simulink library "outp"  (R2021b)
settings: Solver=VariableStepAuto  StartTime=0.0  StopTime=10.0  RelTol=1e-3
undefined symbols (not defined in the file or in its folder): ENUM_PMMMODE_CHARGE, ENUM_PMMMODE_IDLE, ENUM_PMMMODE_INITIALIZE, ENUM_PMMMODE_POWERDOWN, ENUM_PMMMODE_SLEEP, Left, outp, slcm, TRUE
libraries: FVT_lib x686, hcu_lib x4, simulink x1
(part 2 of 7)

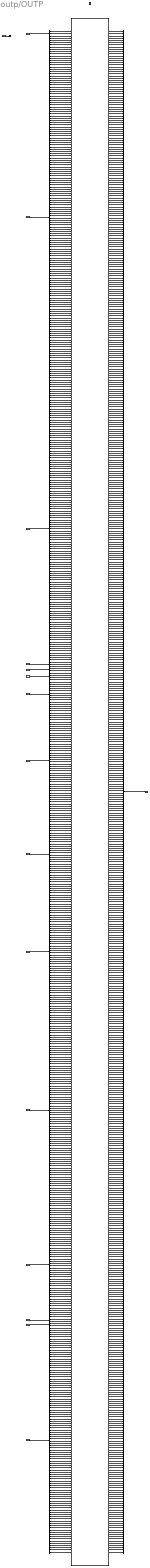
== system outp/OUTP ==
  BACC_outputs : Inport  OutDataTypeStr=Bus: BACC_outputs
  BAPM_outputs : Inport  Port=2  OutDataTypeStr=Bus: BAPM_outputs
  BBCM_outputs : Inport  Port=3  OutDataTypeStr=Bus: BBCM_outputs
  BDDM_outputs : Inport  Port=4
  BDHP_outputs : Inport  Port=5  OutDataTypeStr=Bus: BDHP_outputs
  BDKC_outputs : Inport  Port=6  OutDataTypeStr=Bus: BDKC_outputs
  BDSC_outputs : Inport  Port=7  OutDataTypeStr=Bus: BDSC_outputs
  BNMM_outputs : Inport  Port=8  OutDataTypeStr=Bus: BNMM_outputs
  BPMM_outputs : Inport  Port=9  OutDataTypeStr=Bus: BPMM_outputs
  BSYS_outputs : Inport  Port=10  OutDataTypeStr=Bus: BSYS_outputs
  BTHC_outputs : Inport  Port=11  OutDataTypeStr=Bus: BTHC_outputs
  BTPM_outputs : Inport  Port=12  OutDataTypeStr=Bus: BTPM_outputs
  BTQD_outputs : Inport  Port=13  OutDataTypeStr=Bus: BTQD_outputs
  BTQR_outputs : Inport  Port=14  OutDataTypeStr=Bus: BTQR_outputs
  BV2L_outputs : Inport  Port=15  OutDataTypeStr=Bus: BV2L_outputs
  BVMC_outputs : Inport  Port=16  OutDataTypeStr=Bus: BVMC_outputs
  trig_OUTP : TriggerPort  TriggerType=function-call  VariantControl=(inherit)
  Terminator : Terminator
  bus_creator : BusCreator  Inputs=686
  bus_selector1 : BusSelector  OutputSignals=VACC_HVTHCMSysAvail_enum,VACC_LVBattVoltSta_enum,VACC_VehHVPwrAvail4THCM_W
  bus_selector10 : BusSelector  OutputSignals=VTHC_FDCompCmd_rpm,VTHC_FDSOV1Cmd_flg,VTHC_FDSOV2Cmd_flg,VTHC_FDSOV3Cmd_flg,VTHC_FDEXV1Cmd_step,VTHC_FDEXV2Cmd_step,VTHC_FDSOTXVCmd_flg,VTHC_FDFWVCmd_flg,VTHC_FDTWVCmd_pct,VTHC_FDFrWPTCHeatPwrCmd_W,VTHC_CoolgFanActDuty_pct,VTHC_FDAGSCmd_enum,VTHC_FDEWP1Cmd_enum,VTHC_FDEWP2Cmd_enum,VTHC_FDEWP3Cmd_enum,VTHC_FDFrLeAPTCHeatPwrCmd_W,VTHC_FDFrRiAPTCHeatPwrCmd_W,VTHC_FDRrAPTCHeatPwrCmd_W,VTHC_FDBlowerCmd_pct,VTHC_BatteryMode_enum,VTHC_EDriveMode_enum,VTHC_CabinMode_enum,VTHC_CCUACLampSts_flg,VTHC_CCUAutoLampSts_flg,VTHC_CCUACMaxLampSts_flg,VTHC_CCUSyncLampSts_flg,VTHC_sigAirIntenZon1St_enum,VTHC_sigWindDirZon1St_enum,VTHC_sigRecircSt_flg,VTHC_sigSetTempZon1St_C,VTHC_sigSetTempZon2St_C,VTHC_sigClntTHvBattOut_C,VTHC_sigCbnSolarLeft_W,VTHC_sigClntTHvBattIn_C,VTHC_sigCbnSolarRight_W,VTHC_sigAmbAirT_C,VTHC_sigCbnAirT_C,VTHC_ACSubMode_enum,VTHC_FDRecyAutoCmd_enum,VTHC_ACModeMem_enum,VTHC_Face_flg,VTHC_Foot_flg,VTHC_Frost_flg,VTHC_FaceM_flg,VTHC_FootM_flg,VTHC_CCUSyncSts_flg,VTHC_ACForceOFF_flg,VTHC_RecAutoFlg_flg,VTHC_AirIntenZone1M_enum,VTHC_fdefog_flg,VTHC_sigSetTempZon2StM_C,VTHC_FDCTHCMAPTCWarningSta_flg
  bus_selector11 : BusSelector  OutputSignals=VTPM_LFBatWarn_flg,VTPM_RFBatWarn_flg,VTPM_LRBatWarn_flg,VTPM_RRBatWarn_flg,VTPM_LFWheelPress_raw8,VTPM_RFWheelPress_raw8,VTPM_LRWheelPress_raw8,VTPM_RRWheelPress_raw8,VTPM_LFWheelTemp_C,VTPM_RFWheelTemp_C,VTPM_LRWheelTemp_C,VTPM_RRWheelTemp_C,VTPM_LFSensorFail_flg,VTPM_RFSensorFail_flg,VTPM_LRSensorFail_flg,VTPM_RRSensorFail_flg,VTPM_LFWheelDebug_flg,VTPM_LRWheelDebug_flg,VTPM_RFWheelDebug_flg,VTPM_RRWheelDebug_flg,VTPM_TPMSResButtAllow_flg,VTPM_TPMSCaliButtAllow_flg,VTPM_LFPressIndi_enum,VTPM_RFPressIndi_enum,VTPM_LRPressIndi_enum,VTPM_RRPressIndi_enum,VTPM_TPMSWarnIndi_enum,VTPM_LFWheelTmpIndi_flg,VTPM_RFWheelTmpIndi_flg,VTPM_LRWheelTmpIndi_flg,VTPM_RRWheelTmpIndi_flg,VTPM_LFWheelPSW_raw8,VTPM_LRWheelPSW_raw8,VTPM_RFWheelPSW_raw8,VTPM_RRWheelPSW_raw8,VTPM_CWheelTips_enum,VTPM_AutoLTips_enum,VTPM_LFSensorMode_flg,VTPM_RFSensorMode_flg,VTPM_LRSensorMode_flg,VTPM_RRSensorMode_flg,VTPM_S1ID_raw32,VTPM_S2ID_raw32,VTPM_S3ID_raw32,VTPM_S4ID_raw32,VTPM_S1L_enum,VTPM_S2L_enum,VTPM_S3L_enum,VTPM_S4L_enum,VTPM_ALFin_flg,VTPM_LFP20_raw8,VTPM_RFP20_raw8,VTPM_LRP20_raw8,VTPM_RRP20_raw8,VTPM_FAT_flg,VTPM_IDin_raw32,VTPM_S1WheelDebugALTU_pct,VTPM_S2WheelDebugALTU_pct,VTPM_S3WheelDebugALTU_pct,VTPM_S4WheelDebugALTU_pct,VTPM_ID1messageALTU_raw8,VTPM_ID2messageALTU_raw8,VTPM_ID3messageALTU_raw8,VTPM_ID4messageALTU_raw8,VTPM_Chkfin_flg,VTPM_SetIDLoc_flg,VTPM_TPMSStorge_flg,VTPM_ChkStorge_flg,VTPM_TPMSResButt_flg,VTPM_LFPindi_enum,VTPM_RFPind_enum,VTPM_LRPindi_enum,VTPM_RRPindi_enum,VTPM_WriteChkLFID_raw,VTPM_WriteChkRFID_raw,VTPM_WriteChkLRID_raw,VTPM_WriteChkRRID_raw,VTPM_WriteChkfinLFID_raw,VTPM_WriteChkfinRFID_raw,VTPM_WriteChkfinLRID_raw,VTPM_WriteChkfinRRID_raw,VTPM_Flashchkdatavalid_enum,VTPM_Flashdatavalid_enum,VTPM_unlearnSfali_flg,VTPM_unlearnSfailvalid_enum,VTPM_Prepresstempvalid_enum,VTPM_FlashS1ID_raw,VTPM_FlashS2ID_raw,VTPM_FlashS3ID_raw,VTPM_FlashS4ID_raw,VTPM_FlashIDvalid_enum
  bus_selector12 : BusSelector  OutputSignals=VTQD_ParkRequest_flg,VTQD_TqSourceFr_enum,VTQD_TqSourceRr_enum,VTQD_FrEDUAvailBrkRgnTq_Nm,VTQD_RrEDUAvailBrkRgnTq_Nm,VTQD_EVDriveMode_enum,VTQD_ShiftGearPosn_enum,VTQD_PButtonSta_enum,VTQD_FrActvDmpDisabReq_flg,VTQD_RrActvDmpDisabReq_flg,VTQD_FrRgnDecrSta_flg,VTQD_RrRgnDecrSta_flg,VTQD_DriverWhlTqDemFr_Nm,VTQD_DriverWhlTqDemRr_Nm,VTQD_FrEDUActTq_Nm,VTQD_RrEDUActTq_Nm,VTQD_FrEDURolRgnTq_Nm,VTQD_RrEDURolRgnTq_Nm,VTQD_FrEDUSpd_rpm,VTQD_RrEDUSpd_rpm,VTQD_FrEDUSpdValid_flg,VTQD_FrEDUAvailBrkRgnTqV_flg,VTQD_RrEDUSpdValid_flg,VTQD_RrEDUAvailBrkRgnTqV_flg,VTQD_RgnAbnorSta_flg,VTQD_PTCSPermSta_flg,VTQD_FrRgnPermSta_flg,VTQD_RrRgnPermSta_flg,VTQD_FrIdcMin_A,VTQD_FrIdcMax_A,VTQD_FrUdcMin_V,VTQD_FrUdcMax_V,VTQD_RrIdcMin_A,VTQD_RrIdcMax_A,VTQD_RrUdcMin_V,VTQD_RrUdcMax_V,VTQD_ReBrakeLPReq_flg,VTQD_CreepON_flg,VTQD_EquivAccPedalSWSta_flg,VTQD_DriveProtEn_flg,VTQD_ActParkRequest_flg,VTQD_IVIPwrLockSta_enum,VTQD_OPDHoldLamp_flg,VTQD_SaveRegenMode_enum,VTQD_FDCVCURegenMode_enum,VTQD_SpdCtrlMode_enum,VTQD_SpdCtrlSta_flg,VTQD_SetSpd_kph
  bus_selector13 : BusSelector  OutputSignals=VTQR_FrTMTqReq_Nm,VTQR_RrTMTqReq_Nm
  bus_selector14 : BusSelector  OutputSignals=VV2L_ReqOBCV2LEna_enum,VV2L_ReqV2LIVIPopup_enum
  bus_selector15 : BusSelector  OutputSignals=VVMC_FeatSetSpdFinal_raw32,VVMC_VehicleSpeed_mph,VVMC_VehicleSpeed_kph,VVMC_MeterIndSpeed_raw32,VVMC_VMCAEBCtrlAvail_flg,VVMC_VMCACCCtrlAvail_flg,VVMC_VMCCCCtrlAvail_flg,VVMC_VMCMSACtrlAvail_flg,VVMC_FeatArbitrSta_enum,VVMC_FeatReqSpd_kph,VVMC_JerkPCT_pct,VVMC_LimitPCT_pct,VVMC_FrontRearSlipRatioCtrl_flg,VVMC_RearWhlSlipRatioCtrl_flg,VVMC_SingleWhlSlipRatioCtrl_flg,VVMC_LatAccCtrl_flg,VVMC_SafetyCtrl_flg,VVMC_SPD2ACCAct_flg,VVMC_AccCalcuPID_mps2,VVMC_ISOAccLimit_mps2,VVMC_ISODecLimit_mps2,VVMC_ISOJerkLimit_mps3,VVMC_ACCRequiredAccel_mps2,VVMC_DISCReqAcc_mps2,VVMC_FeatArbitrFinal_enum,VVMC_LateralCtrl_flg,VVMC_ADASLKASta_enum,VVMC_LKAStrToqReq_Nm,VVMC_LKATOIFault_flg,VVMC_LKATOIAct_enum,VVMC_ADASAEBReq_enum,VVMC_ADASFaultSta_flg,VVMC_AEBVehHoldReq_flg,VVMC_ACCVehHoldReq_flg,VVMC_ADASDBSReq_enum,VVMC_ADASACCSta_enum,VVMC_ACCObjDist_m,VVMC_ACCObjRelSpd_mps,VVMC_TimeGapLevel_enum,VVMC_ACCJerkUpperLimit_mps3,VVMC_ACCComfortBandUpper_mps2,VVMC_ACCJerkLowerLimit_mps3,VVMC_ACCComfortBandLower_mps2,VVMC_ADASVehSpdLim_raw32,VVMC_ADASShftPosnReqA_flg,VVMC_ADASShftPosnReq_enum,VVMC_ADASForceIdle_flg,VVMC_HazardWarningReq_flg,VVMC_RightTurnLightReq_flg,VVMC_LeftTurnLightReq_flg,VVMC_ADASFCWSta_enum,VVMC_ADASLDWSta_enum,VVMC_ADASFltWrnReq_flg,VVMC_ACCObjDstLvl_enum,VVMC_ForceLowBeam_enum,VVMC_ACCTakeoverReq_flg,VVMC_ADASWarningMsg_enum,VVMC_ADASCAMSpdLim_enum,VVMC_TargetType_enum,VVMC_ADASSLIFSpdLim_enum,VVMC_LKAHODDisplayWarning_flg,VVMC_LKAHODSoundWarning_flg,VVMC_ADASLFCSta_enum,VVMC_ADASLaneModeL_enum,VVMC_ADASLaneModeR_enum,VVMC_ADASSLIFSta_enum,VVMC_ADASISASta_enum,VVMC_ADASLDWMute_flg,VVMC_ADASFCWMute_flg,VVMC_ADASLFCHandsOffWarning_enum,VVMC_LVDADisabled_flg,VVMC_LVDAMuteSta_enum,VVMC_LVDAFailinfo_flg,VVMC_LVDAWarning_flg,VVMC_LVDAACCStatusInformation_flg,VVMC_ADASLFCWarnSound_enum,VVMC_FCMACCmode_enum,VVMC_ADASLanetypeR_enum,VVMC_ADASLanetypeL_enum,VVMC_ADASLanecurveL_raw32,VVMC_ADASLanecurveR_raw32,VVMC_ADASAEBSta_enum,VVMC_FCMLDWRequest_enum,VVMC_FCMLDWFault_flg,VVMC_ACCCtrlAvail_flg,VVMC_ACCPedalOvrd_flg,VVMC_TimeGapCalcu_s,VVMC_CCCtrlSta_enum,VVMC_MSACtrlSta_enum,VVMC_APSCtrlAvail_flg,VVMC_APSStaSys_enum,VVMC_APSDecReqA_flg,VVMC_APSDecReq_mps2,VVMC_APSReq_enum,VVMC_CCMSASpdWar_flg,VVMC_IMUEnaCmd_flg,VVMC_CAASCtrlAvail_flg,VVMC_CAASActive_flg,VVMC_VMCRWSActvSta_enum,VVMC_VMCRWSDfctvSta_enum,VVMC_VMCRWSPositionReq_mm,VVMC_VMCSteerFaultRequest_enum
  bus_selector2 : BusSelector  OutputSignals=VAPM_VehSpeed_kph,VAPM_VehSpeedTimeOut_flg,VAPM_FSOffSw_enum,VAPM_FSOffSwTimeOut_flg,VAPM_ChrgPlugSta_enum,VAPM_PASDRMR_cm,VAPM_PASDRML_cm,VAPM_PASDRCR_cm,VAPM_PASDRCL_cm,VAPM_PASDFMR_cm,VAPM_PASDFML_cm,VAPM_PASDFCR_cm,VAPM_PASDFCL_cm,VAPM_APSDRLR_cm,VAPM_APSDRLL_cm,VAPM_APSDFLR_cm,VAPM_APSDFLL_cm,VAPM_PASAFCL_enum,VAPM_PASARMR_enum,VAPM_PASARML_enum,VAPM_PASARCR_enum,VAPM_PASARCL_enum,VAPM_PASAFMR_enum,VAPM_PASAFML_enum,VAPM_PASAFCR_enum,VAPM_USSStaRMR_flg,VAPM_USSStaRML_flg,VAPM_USSStaRLR_flg,VAPM_USSStaRLL_flg,VAPM_USSStaRCR_flg,VAPM_USSStaRCL_flg,VAPM_USSStaFMR_flg,VAPM_USSStaFML_flg,VAPM_USSStaFLR_flg,VAPM_USSStaFLL_flg,VAPM_USSStaFCR_flg,VAPM_USSStaFCL_flg,VAPM_Chime_enum,VAPM_SNSRLayout_enum,VAPM_StaFSya_flg,VAPM_ModOperation_enum,VAPM_BrkPedalPos_pct,VAPM_BrkPedalPosTimeOut_flg,VAPM_LFRawWhlSpeed_kph,VAPM_LFRawWhlSpeedTimeOut_flg,VAPM_RFRawWhlSpeed_kph,VAPM_RFRawWhlSpeedTimeOut_flg,VAPM_LRRawWhlSpeed_kph,VAPM_LRRawWhlSpeedTimeOut_flg,VAPM_RRRawWhlSpeed_kph,VAPM_RRRawWhlSpeedTimeOut_flg,VAPM_LFRawWhlSpeedV_flg,VAPM_LFRawWhlSpeedVTimeOut_flg,VAPM_RFRawWhlSpeedV_flg,VAPM_RFRawWhlSpeedVTimeOut_flg,VAPM_LRRawWhlSpeedV_flg,VAPM_LRRawWhlSpeedVTimeOut_flg,VAPM_RRRawWhlSpeedV_flg,VAPM_RRRawWhlSpeedVTimeOut_flg,VAPM_LFWhlRotDir_enum,VAPM_LFWhlRotDirTimeOut_flg,VAPM_RFWhlRotDir_enum,VAPM_RFWhlRotDirTimeOut_flg,VAPM_LRWhlRotDir_enum,VAPM_LRWhlRotDirTimeOut_flg,VAPM_RRWhlRotDir_enum,VAPM_RRWhlRotDirTimeOut_flg,VAPM_LFPulseCountV_flg,VAPM_LFPulseCountVTimeOut_flg,VAPM_RFPulseCountV_flg,VAPM_RFPulseCountVTimeOut_flg,VAPM_LRPulseCountV_flg,VAPM_LRPulseCountVTimeOut_flg,VAPM_RRPulseCountV_flg,VAPM_RRPulseCountVTimeOut_flg,VAPM_LFPulseCount_enum,VAPM_LFPulseCountTimeOut_flg,VAPM_RFPulseCount_enum,VAPM_RFPulseCountTimeOut_flg,VAPM_LRPulseCount_enum,VAPM_LRPulseCountTimeOut_flg,VAPM_RRPulseCount_enum,VAPM_RRPulseCountTimeOut_flg,VAPM_ShifterHandleCmd_enum,VAPM_ShifterHandleCmdTimeOut_flg,VAPM_DriIntend_enum,VAPM_DriIntendTimeOut_flg,VAPM_EPSAOIControl_enum,VAPM_EPSAOIControlTimeOut_flg,VAPM_SASAngle_Deg,VAPM_SASAngleTimeOut_flg,VAPM_SASSpeed_degps,VAPM_SASSpeedTimeOut_flg,VAPM_SASSpeedValid_flg,VAPM_SASSpeedValidTimeOut_flg,VAPM_SASCAL_flg,VAPM_SASCALTimeOut_flg,VAPM_SASV_flg,VAPM_SASVTimeOut_flg,VAPM_GRADE_Deg,VAPM_GRADETimeOut_flg,VAPM_YawRate_degps,VAPM_YawRateTimeOut_flg,VAPM_LatAccel_Gps,VAPM_LatAccelTimeOut_flg,VAPM_LongAccel_Gps,VAPM_LongAccelTimeOut_flg,VAPM_MCPressure_bar,VAPM_MCPressureTimeOut_flg,VAPM_YawRateV_flg,VAPM_YawRateVTimeOut_flg,VAPM_LatAccelV_flg,VAPM_LatAccelVTimeOut_flg,VAPM_LongAccelV_flg,VAPM_LongAccelVTimeOut_flg,VAPM_MCPressureV_bar,VAPM_MCPressureVTimeOut_flg,VAPM_BrkSwSta_flg,VAPM_BrkSwStaTimeOut_flg,VAPM_BrkSwV_flg,VAPM_BrkSwVTimeOut_flg,VAPM_ESCStandstill_flg,VAPM_ESCStandstillTimeOut_flg,VAPM_ESCAPSSta_enum,VAPM_ESCAPSStaTimeOut_flg,VAPM_EPBExtReleaseAvail_flg,VAPM_EPBExtReleaseAvailTimeOut_flg,VAPM_EPBExtApplyAvail_flg,VAPM_EPBExtApplyAvailTimeOut_flg,VAPM_EPBErrSta_enum,VAPM_EPBErrStaTimeOut_flg,VAPM_EPBSta_enum,VAPM_EPBStaTimeOut_flg,VAPM_AVMparkingcancel_enum,VAPM_AVMparkingcancelTimeOut_flg,VAPM_AVMparkingexcute_enum,VAPM_AVMparkingexcuteTimeOut_flg,VAPM_AVMParkingmode_enum,VAPM_AVMParkingmodeTimeOut_flg,VAPM_AVMErrSTA_flg,VAPM_AVMErrSTATimeOut_flg,VAPM_IVIStatus_flg,VAPM_IVIStatusTimeOut_flg,VAPM_CAASSw_enum,VAPM_CAASSwTimeOut_flg,VAPM_IVIScreen_enum,VAPM_IVIScreenTimeOut_flg,VAPM_ABSActive_flg,VAPM_ABSActiveTimeOut_flg,VAPM_TCSActive_flg,VAPM_TCSActiveTimeOut_flg,VAPM_DriverSeatBeltCmd_flg,VAPM_DriverSeatBeltCmdTimeOut_flg,VAPM_APSProgressPCT_pct,VAPM_APSRQDisplay_enum,VAPM_APSSWVer_enum,VAPM_APSHWVer_enum,VAPM_APSExitCondition_enum,VAPM_APSAngleTarget_Deg,VAPM_APSVRqEPASCtrl_flg,VAPM_APSRqEPASCtrl_flg,VAPM_CAASSta_enum
  bus_selector3 : BusSelector  OutputSignals=VBCM_AntitheftSta_enum,VBCM_TailgateRemote_enum,VBCM_HornCtrl_flg,VBCM_AllDoorSW_flg,VBCM_BCMDoorLockSta_flg,VBCM_AntitheftSeatFlod_flg,VBCM_HoodSW_flg,VBCM_TailgateSW_flg,VBCM_DrDoorSW_flg,VBCM_PsDoorSW_flg,VBCM_RLDoorSW_flg,VBCM_RRDoorSW_flg,VBCM_LockSetting_flg,VBCM_FrChargingDoorCtrl_enum,VBCM_RrChargingDoorCtrl_enum,VBCM_CrashDetd_flg,VBCM_CTDCtrl_enum,VBCM_DoorLockIND_flg,VBCM_CTDLockSW_flg,VBCM_Dimmer_pct,VBCM_DimmerEN_flg,VBCM_PosLamp_flg,VBCM_LBeam_flg,VBCM_HBeam_flg,VBCM_RrFogLamp_flg,VBCM_BrakeLamp_flg,VBCM_ReverseLamp_flg,VBCM_LDRL_flg,VBCM_RDRL_flg,VBCM_LBSD_flg,VBCM_RBSD_flg,VBCM_HazardSW_flg,VBCM_LTurnLP_flg,VBCM_RTurnLP_flg,VBCM_BCMBuzzerReq_flg,VBCM_MirrorCtrl_enum,VBCM_MirrorDefog_flg,VBCM_RrDefog_flg,VBCM_RoomLampH_flg,VBCM_RoomLampL_flg,VBCM_TrunkRel_flg,VBCM_TailgateHDSW_flg,VBCM_FrWiperL_flg,VBCM_FrWiperH_flg,VBCM_RrWiper_flg,VBCM_WasherCtrl_enum,VBCM_WiperFixMode_flg,VBCM_AmbLightBreath1_enum,VBCM_AmbLightBreath2_enum,VBCM_AmbLightBreath3_enum,VBCM_AmbLightBreath4_enum,VBCM_AmbLightBreath5_enum,VBCM_AmbLightBreath6_enum,VBCM_AmbLightBrightness1_enum,VBCM_AmbLightBrightness2_enum,VBCM_AmbLightBrightness3_enum,VBCM_AmbLightBrightness4_enum,VBCM_AmbLightBrightness5_enum,VBCM_AmbLightBrightness6_enum,VBCM_AmbLightColor1_enum,VBCM_AmbLightColor2_enum,VBCM_AmbLightColor3_enum,VBCM_AmbLightColor4_enum,VBCM_AmbLightColor5_enum,VBCM_AmbLightColor6_enum,VBCM_LampPwr_flg,VBCM_SPTGDet_flg,VBCM_APSOpenPTG_flg,VBCM_FollowMe_flg,VBCM_IVIRST_flg,VBCM_CountAlarm_enum,VBCM_MFSWTri_flg,VBCM_MirrorFlodPos_flg,VBCM_FuelDoorPos_flg,VBCM_MFRDNBrightReq_pct,VBCM_RoomLampMode_flg,VBCM_IVIPTGUSStaSW_flg,VBCM_PTGInnerSW2_enum,VBCM_LDrvCtrlCmd_pct,VBCM_LPasCtrlCmd_pct,VBCM_LRLDCtrlCmd_pct,VBCM_LRRDCtrlCmd_pct,VBCM_APMDoorControlSta_flg,VBCM_AmbFunEN_flg,VBCM_AmbWelEN_flg,VBCM_AmbDimEN_flg,VBCM_AmbLinkDriSta_flg,VBCM_AmbPwrWarnEN_flg,VBCM_AmbODAEN_flg,VBCM_AmbColorSta_enum,VBCM_AmbBrightSta_enum,VBCM_LockAlarm_enum,VBCM_ATCtrl_enum,VBCM_fUnlockSingle_flg,VBCM_UserNow_enum,VBCM_AmbFunENFlash_enum,VBCM_AmbWelENFlash_enum,VBCM_AmbDimENFlash_enum,VBCM_AmbLinkDriStaFlash_enum,VBCM_AmbPwrWarnENFlash_enum,VBCM_AmbODAENFlash_enum,VBCM_AmbColorSta1_enum,VBCM_AmbColorSta2_enum,VBCM_AmbColorSta3_enum,VBCM_AmbColorSta4_enum,VBCM_AmbColorSta5_enum,VBCM_AmbColorSta7_enum,VBCM_AmbBrightnessSta1_enum,VBCM_AmbBrightnessSta2_enum,VBCM_AmbBrightnessSta3_enum,VBCM_AmbBrightnessSta4_enum,VBCM_AmbBrightnessSta5_enum,VBCM_AmbBrightnessSta7_enum,VBCM_HazardIND_flg,VBCM_DimSwSta_flg,VBCM_PassSWSta_flg,VBCM_FWipSwSta_enum,VBCM_FWasSwSta_enum,VBCM_TurnSwSta_enum
  bus_selector4 : BusSelector  OutputSignals=VDHP_ActAPSPosn_pct,VDHP_EAPS1MIN_pct,VDHP_EAPS2MIN_pct
  bus_selector5 : BusSelector  OutputSignals=VDKC_DKCTimeSN_cnt,VDKC_DKCAuthSta_enum
  bus_selector6 : BusSelector  OutputSignals=VDSC_DISCTurn_flg,VDSC_DISCTargetSpd_kph,VDSC_DISCSta_enum,VDSC_DISCButtSta_flg
  bus_selector7 : BusSelector  OutputSignals=VNMM_AllCANTxReq_flg,VNMM_NMmTxReq_flg,VNMM_Awake_enum,VNMM_CSB_flg,VNMM_ErrorState_enum,VNMM_NodeID_enum,VNMM_PNI_flg,VNMM_RptMsgReq_flg,VNMM_WakeUp_enum,VNMM_ActiveWU_flg,VNMM_SysNMmSta_enum,VNMM_NetworkReq_flg
  bus_selector8 : BusSelector  OutputSignals=VPMM_PowerUpState_enum,VPMM_PowerDownState_enum,VPMM_PowerUpFault_enum,VPMM_PowerDownFault_enum,VPMM_ActiveDischargeReq_flg,VPMM_DCDCEnaReq_flg,VPMM_DCDCVoltSetpoint_V,VPMM_HVBatCnctReq_flg,VPMM_HVSysReadyToCharge_enum,VPMM_PowerSta_enum,VPMM_LVPwrSta_flg,VPMM_HVPwrSta_flg,VPMM_SysPowerMode_enum,VPMM_FrMCUEnaReq_flg,VPMM_RrMCUEnaReq_flg,VPMM_DrivetrainSelect_enum,VPMM_DrSeatSta_enum,VPMM_PwrStaSelect_enum,VPMM_PwrStaConstraint_enum,VPMM_TCountSta_enum,VPMM_PwrUpReq_enum,VPMM_PwrDownReq_enum,VPMM_LowSOCWarn_enum,VPMM_ReVehThdChkSta_enum,VPMM_LVSysErrPwrOutErr_flg,VPMM_EvccAplusPwrUpReq_flg,VPMM_PwrStaONTOPopReq_flg,VPMM_IVIPwrStaONTOPopT_s,VPMM_LVChrgHoldTtimer_s,VPMM_LVBattChrgTimeCnt_s,VPMM_SilentChkAllowSleep_flg,VPMM_TimerAllowSleep_flg,VPMM_FDADC12VDetAvg_mV,VPMM_PMMAllowECUSleep_flg,VPMM_LVSilentChrgSta_enum,VPMM_LVSilentChrgReq_flg,VPMM_LVSilentChrgLv_enum,VPMM_CtrlFrPwrStbA1P_flg,VPMM_CtrlFrRC1_flg,VPMM_CtrlFrBMSCCUCIR_flg,VPMM_CtrlFrEDUINVERTER_flg,VPMM_HWResetSta_enum,VPMM_CtrlDrPwrStbA2_flg,VPMM_PwrStaTOSta_enum,VPMM_Sched_ChgTOSta_enum,VPMM_PwrReq_OTA_enum,VPMM_OTAPwrReqOFFChkSta_enum,VPMM_OTAPwrReqStdChkSta_enum
  bus_selector9 : BusSelector  OutputSignals=VSYS_HWVer1_cnt,VSYS_HWVer2_cnt,VSYS_HWVer3_cnt,VSYS_CarModel1_cnt,VSYS_CarModel2_cnt,VSYS_CarModel3_cnt,VSYS_ECU1_cnt,VSYS_ECU2_cnt,VSYS_Major1_cnt,VSYS_Major2_cnt,VSYS_Minor1_cnt,VSYS_Minor2_cnt,VSYS_Patch1_cnt,VSYS_Patch2_cnt,VSYS_Country1_cnt,VSYS_Country2_cnt,VSYS_Variation_cnt,VSYS_Dash1_cnt,VSYS_Change1_cnt,VSYS_Change2_cnt,VSYS_Dash2_cnt,VSYS_SHA1_cnt,VSYS_SHA2_cnt,VSYS_SHA3_cnt,VSYS_SHA4_cnt,VSYS_SHA5_cnt,VSYS_SHA6_cnt,VSYS_SHA7_cnt,VSYS_SHA8_cnt,VSYS_NvWriteReqRisingEdge_flg,VSYS_FdcSlpReqRisingEdge_flg,VSYS_FdcSlpTime_sec,VSYS_PmicBootReason_enum,VSYS_WisrBootReason_raw32,VSYS_AcoreRebootCmdACK_flg,VSYS_CurrentNmState_enum
  outpmodule : Subsystem
  BOUTP_outputs : Outport  OutDataTypeStr=Bus: BOUTP_outputs
  wires:
  BDDM_outputs/1 -> Terminator/1
  outpmodule/92(VOUTP_EPSAOIControlTimeOut_flg) -> bus_creator/92
  outpmodule/91(VOUTP_EPSAOIControl_enum) -> bus_creator/91
  outpmodule/90(VOUTP_DriIntendTimeOut_flg) -> bus_creator/90
  outpmodule/117(VOUTP_LongAccelV_flg) -> bus_creator/117
  outpmodule/87(VOUTP_ShifterHandleCmd_enum) -> bus_creator/87
  bus_selector15/101 -> outpmodule/685(VVMC_VMCRWSPositionReq_mm)  "<VVMC_VMCRWSPositionReq_mm>"
  bus_selector15/102 -> outpmodule/686(VVMC_VMCSteerFaultRequest_enum)  "<VVMC_VMCSteerFaultRequest_enum>"
  bus_selector15/100 -> outpmodule/684(VVMC_VMCRWSDfctvSta_enum)  "<VVMC_VMCRWSDfctvSta_enum>"
  outpmodule/97(VOUTP_SASSpeedValid_flg) -> bus_creator/97
  bus_selector15/97 -> outpmodule/681(VVMC_CAASCtrlAvail_flg)  "<VVMC_CAASCtrlAvail_flg>"
  bus_selector15/95 -> outpmodule/679(VVMC_CCMSASpdWar_flg)  "<VVMC_CCMSASpdWar_flg>"
  bus_selector15/94 -> outpmodule/678(VVMC_APSReq_enum)  "<VVMC_APSReq_enum>"
  bus_selector15/92 -> outpmodule/676(VVMC_APSDecReqA_flg)  "<VVMC_APSDecReqA_flg>"
  bus_selector15/89 -> outpmodule/673(VVMC_MSACtrlSta_enum)  "<VVMC_MSACtrlSta_enum>"
  bus_selector15/86 -> outpmodule/670(VVMC_ACCPedalOvrd_flg)  "<VVMC_ACCPedalOvrd_flg>"
  bus_selector15/85 -> outpmodule/669(VVMC_ACCCtrlAvail_flg)  "<VVMC_ACCCtrlAvail_flg>"
  bus_selector15/79 -> outpmodule/663(VVMC_ADASLanetypeL_enum)  "<VVMC_ADASLanetypeL_enum>"
  bus_selector15/80 -> outpmodule/664(VVMC_ADASLanecurveL_raw32)  "<VVMC_ADASLanecurveL_raw32>"
  bus_selector15/78 -> outpmodule/662(VVMC_ADASLanetypeR_enum)  "<VVMC_ADASLanetypeR_enum>"
  bus_selector15/77 -> outpmodule/661(VVMC_FCMACCmode_enum)  "<VVMC_FCMACCmode_enum>"
  bus_selector15/76 -> outpmodule/660(VVMC_ADASLFCWarnSound_enum)  "<VVMC_ADASLFCWarnSound_enum>"
  bus_selector15/75 -> outpmodule/659(VVMC_LVDAACCStatusInformation_flg)  "<VVMC_LVDAACCStatusInformation_flg>"
  bus_selector15/74 -> outpmodule/658(VVMC_LVDAWarning_flg)  "<VVMC_LVDAWarning_flg>"
  bus_selector15/69 -> outpmodule/653(VVMC_ADASFCWMute_flg)  "<VVMC_ADASFCWMute_flg>"
  bus_selector15/67 -> outpmodule/651(VVMC_ADASISASta_enum)  "<VVMC_ADASISASta_enum>"
  bus_selector15/66 -> outpmodule/650(VVMC_ADASSLIFSta_enum)  "<VVMC_ADASSLIFSta_enum>"
  bus_selector15/65 -> outpmodule/649(VVMC_ADASLaneModeR_enum)  "<VVMC_ADASLaneModeR_enum>"
  outpmodule/95(VOUTP_SASSpeed_degps) -> bus_creator/95
  bus_selector15/63 -> outpmodule/647(VVMC_ADASLFCSta_enum)  "<VVMC_ADASLFCSta_enum>"
  bus_selector15/60 -> outpmodule/644(VVMC_ADASSLIFSpdLim_enum)  "<VVMC_ADASSLIFSpdLim_enum>"
  bus_selector15/59 -> outpmodule/643(VVMC_TargetType_enum)  "<VVMC_TargetType_enum>"
  bus_selector15/55 -> outpmodule/639(VVMC_ForceLowBeam_enum)  "<VVMC_ForceLowBeam_enum>"
  bus_selector15/51 -> outpmodule/635(VVMC_ADASFCWSta_enum)  "<VVMC_ADASFCWSta_enum>"
  bus_selector15/53 -> outpmodule/637(VVMC_ADASFltWrnReq_flg)  "<VVMC_ADASFltWrnReq_flg>"
  bus_selector15/52 -> outpmodule/636(VVMC_ADASLDWSta_enum)  "<VVMC_ADASLDWSta_enum>"
  bus_selector15/50 -> outpmodule/634(VVMC_LeftTurnLightReq_flg)  "<VVMC_LeftTurnLightReq_flg>"
  bus_selector15/49 -> outpmodule/633(VVMC_RightTurnLightReq_flg)  "<VVMC_RightTurnLightReq_flg>"
  bus_selector15/48 -> outpmodule/632(VVMC_HazardWarningReq_flg)  "<VVMC_HazardWarningReq_flg>"
  bus_selector15/73 -> outpmodule/657(VVMC_LVDAFailinfo_flg)  "<VVMC_LVDAFailinfo_flg>"
  bus_selector15/46 -> outpmodule/630(VVMC_ADASShftPosnReq_enum)  "<VVMC_ADASShftPosnReq_enum>"
  bus_selector15/43 -> outpmodule/627(VVMC_ACCComfortBandLower_mps2)  "<VVMC_ACCComfortBandLower_mps2>"
  bus_selector15/41 -> outpmodule/625(VVMC_ACCComfortBandUpper_mps2)  "<VVMC_ACCComfortBandUpper_mps2>"
  bus_selector15/42 -> outpmodule/626(VVMC_ACCJerkLowerLimit_mps3)  "<VVMC_ACCJerkLowerLimit_mps3>"
  outpmodule/93(VOUTP_SASAngle_Deg) -> bus_creator/93
  bus_selector15/29 -> outpmodule/613(VVMC_LKATOIFault_flg)  "<VVMC_LKATOIFault_flg>"
  bus_selector15/19 -> outpmodule/603(VVMC_AccCalcuPID_mps2)  "<VVMC_AccCalcuPID_mps2>"
  bus_selector15/17 -> outpmodule/601(VVMC_SafetyCtrl_flg)  "<VVMC_SafetyCtrl_flg>"
  bus_selector15/18 -> outpmodule/602(VVMC_SPD2ACCAct_flg)  "<VVMC_SPD2ACCAct_flg>"
  bus_selector15/33 -> outpmodule/617(VVMC_AEBVehHoldReq_flg)  "<VVMC_AEBVehHoldReq_flg>"
  bus_selector15/15 -> outpmodule/599(VVMC_SingleWhlSlipRatioCtrl_flg)  "<VVMC_SingleWhlSlipRatioCtrl_flg>"
  bus_selector15/14 -> outpmodule/598(VVMC_RearWhlSlipRatioCtrl_flg)  "<VVMC_RearWhlSlipRatioCtrl_flg>"
  bus_selector15/37 -> outpmodule/621(VVMC_ACCObjDist_m)  "<VVMC_ACCObjDist_m>"
  bus_selector15/13 -> outpmodule/597(VVMC_FrontRearSlipRatioCtrl_flg)  "<VVMC_FrontRearSlipRatioCtrl_flg>"
  bus_selector15/12 -> outpmodule/596(VVMC_LimitPCT_pct)  "<VVMC_LimitPCT_pct>"
  bus_selector15/10 -> outpmodule/594(VVMC_FeatReqSpd_kph)  "<VVMC_FeatReqSpd_kph>"
  bus_selector15/8 -> outpmodule/592(VVMC_VMCMSACtrlAvail_flg)  "<VVMC_VMCMSACtrlAvail_flg>"
  bus_selector15/11 -> outpmodule/595(VVMC_JerkPCT_pct)  "<VVMC_JerkPCT_pct>"
  bus_selector15/32 -> outpmodule/616(VVMC_ADASFaultSta_flg)  "<VVMC_ADASFaultSta_flg>"
  bus_selector15/5 -> outpmodule/589(VVMC_VMCAEBCtrlAvail_flg)  "<VVMC_VMCAEBCtrlAvail_flg>"
  bus_selector15/9 -> outpmodule/593(VVMC_FeatArbitrSta_enum)  "<VVMC_FeatArbitrSta_enum>"
  bus_selector15/1 -> outpmodule/585(VVMC_FeatSetSpdFinal_raw32)  "<VVMC_FeatSetSpdFinal_raw32>"
  bus_selector14/1 -> outpmodule/583(VV2L_ReqOBCV2LEna_enum)  "<VV2L_ReqOBCV2LEna_enum>"
  BV2L_outputs/1 -> bus_selector14/1
  bus_selector13/1 -> outpmodule/581(VTQR_FrTMTqReq_Nm)  "<VTQR_FrTMTqReq_Nm>"
  BTQD_outputs/1 -> bus_selector12/1
  bus_selector13/2 -> outpmodule/582(VTQR_RrTMTqReq_Nm)  "<VTQR_RrTMTqReq_Nm>"
  bus_selector12/48 -> outpmodule/580(VTQD_SetSpd_kph)  "<VTQD_SetSpd_kph>"
  bus_selector12/47 -> outpmodule/579(VTQD_SpdCtrlSta_flg)  "<VTQD_SpdCtrlSta_flg>"
  bus_selector12/42 -> outpmodule/574(VTQD_IVIPwrLockSta_enum)  "<VTQD_IVIPwrLockSta_enum>"
  bus_selector12/43 -> outpmodule/575(VTQD_OPDHoldLamp_flg)  "<VTQD_OPDHoldLamp_flg>"
  bus_selector11/32 -> outpmodule/473(VTPM_LFWheelPSW_raw8)  "<VTPM_LFWheelPSW_raw8>"
  bus_selector11/31 -> outpmodule/472(VTPM_RRWheelTmpIndi_flg)  "<VTPM_RRWheelTmpIndi_flg>"
  bus_selector11/30 -> outpmodule/471(VTPM_LRWheelTmpIndi_flg)  "<VTPM_LRWheelTmpIndi_flg>"
  bus_selector11/46 -> outpmodule/487(VTPM_S1L_enum)  "<VTPM_S1L_enum>"
  bus_selector11/29 -> outpmodule/470(VTPM_RFWheelTmpIndi_flg)  "<VTPM_RFWheelTmpIndi_flg>"
  bus_selector11/27 -> outpmodule/468(VTPM_TPMSWarnIndi_enum)  "<VTPM_TPMSWarnIndi_enum>"
  BTHC_outputs/1 -> bus_selector10/1
  bus_selector10/51 -> outpmodule/440(VTHC_sigSetTempZon2StM_C)  "<VTHC_sigSetTempZon2StM_C>"
  bus_selector10/52 -> outpmodule/441(VTHC_FDCTHCMAPTCWarningSta_flg)  "<VTHC_FDCTHCMAPTCWarningSta_flg>"
  bus_selector10/50 -> outpmodule/439(VTHC_fdefog_flg)  "<VTHC_fdefog_flg>"
  bus_selector10/49 -> outpmodule/438(VTHC_AirIntenZone1M_enum)  "<VTHC_AirIntenZone1M_enum>"
  bus_selector10/47 -> outpmodule/436(VTHC_ACForceOFF_flg)  "<VTHC_ACForceOFF_flg>"
  bus_selector10/45 -> outpmodule/434(VTHC_FootM_flg)  "<VTHC_FootM_flg>"
  bus_selector10/46 -> outpmodule/435(VTHC_CCUSyncSts_flg)  "<VTHC_CCUSyncSts_flg>"
  bus_selector10/43 -> outpmodule/432(VTHC_Frost_flg)  "<VTHC_Frost_flg>"
  bus_selector10/40 -> outpmodule/429(VTHC_ACModeMem_enum)  "<VTHC_ACModeMem_enum>"
  bus_selector10/44 -> outpmodule/433(VTHC_FaceM_flg)  "<VTHC_FaceM_flg>"
  bus_selector10/42 -> outpmodule/431(VTHC_Foot_flg)  "<VTHC_Foot_flg>"
  bus_selector10/37 -> outpmodule/426(VTHC_sigCbnAirT_C)  "<VTHC_sigCbnAirT_C>"
  bus_selector10/35 -> outpmodule/424(VTHC_sigCbnSolarRight_W)  "<VTHC_sigCbnSolarRight_W>"
  bus_selector10/34 -> outpmodule/423(VTHC_sigClntTHvBattIn_C)  "<VTHC_sigClntTHvBattIn_C>"
  bus_selector10/32 -> outpmodule/421(VTHC_sigClntTHvBattOut_C)  "<VTHC_sigClntTHvBattOut_C>"
  bus_selector10/33 -> outpmodule/422(VTHC_sigCbnSolarLeft_W)  "<VTHC_sigCbnSolarLeft_W>"
  bus_selector10/31 -> outpmodule/420(VTHC_sigSetTempZon2St_C)  "<VTHC_sigSetTempZon2St_C>"
  bus_selector10/30 -> outpmodule/419(VTHC_sigSetTempZon1St_C)  "<VTHC_sigSetTempZon1St_C>"
  bus_selector10/28 -> outpmodule/417(VTHC_sigWindDirZon1St_enum)  "<VTHC_sigWindDirZon1St_enum>"
  bus_selector10/27 -> outpmodule/416(VTHC_sigAirIntenZon1St_enum)  "<VTHC_sigAirIntenZon1St_enum>"
  bus_selector10/24 -> outpmodule/413(VTHC_CCUAutoLampSts_flg)  "<VTHC_CCUAutoLampSts_flg>"
  bus_selector10/26 -> outpmodule/415(VTHC_CCUSyncLampSts_flg)  "<VTHC_CCUSyncLampSts_flg>"
  bus_selector10/25 -> outpmodule/414(VTHC_CCUACMaxLampSts_flg)  "<VTHC_CCUACMaxLampSts_flg>"
  bus_selector10/23 -> outpmodule/412(VTHC_CCUACLampSts_flg)  "<VTHC_CCUACLampSts_flg>"
  bus_selector10/22 -> outpmodule/411(VTHC_CabinMode_enum)  "<VTHC_CabinMode_enum>"
  bus_selector10/21 -> outpmodule/410(VTHC_EDriveMode_enum)  "<VTHC_EDriveMode_enum>"
  bus_selector10/19 -> outpmodule/408(VTHC_FDBlowerCmd_pct)  "<VTHC_FDBlowerCmd_pct>"
  bus_selector10/15 -> outpmodule/404(VTHC_FDEWP3Cmd_enum)  "<VTHC_FDEWP3Cmd_enum>"
  bus_selector10/12 -> outpmodule/401(VTHC_FDAGSCmd_enum)  "<VTHC_FDAGSCmd_enum>"
  bus_selector10/13 -> outpmodule/402(VTHC_FDEWP1Cmd_enum)  "<VTHC_FDEWP1Cmd_enum>"
  bus_selector10/10 -> outpmodule/399(VTHC_FDFrWPTCHeatPwrCmd_W)  "<VTHC_FDFrWPTCHeatPwrCmd_W>"
  bus_selector10/8 -> outpmodule/397(VTHC_FDFWVCmd_flg)  "<VTHC_FDFWVCmd_flg>"
  bus_selector10/6 -> outpmodule/395(VTHC_FDEXV2Cmd_step)  "<VTHC_FDEXV2Cmd_step>"
  bus_selector10/16 -> outpmodule/405(VTHC_FDFrLeAPTCHeatPwrCmd_W)  "<VTHC_FDFrLeAPTCHeatPwrCmd_W>"
  bus_selector11/37 -> outpmodule/478(VTPM_AutoLTips_enum)  "<VTPM_AutoLTips_enum>"
  bus_selector10/4 -> outpmodule/393(VTHC_FDSOV3Cmd_flg)  "<VTHC_FDSOV3Cmd_flg>"
  bus_selector10/3 -> outpmodule/392(VTHC_FDSOV2Cmd_flg)  "<VTHC_FDSOV2Cmd_flg>"
  bus_selector11/24 -> outpmodule/465(VTPM_RFPressIndi_enum)  "<VTPM_RFPressIndi_enum>"
  bus_selector11/22 -> outpmodule/463(VTPM_TPMSCaliButtAllow_flg)  "<VTPM_TPMSCaliButtAllow_flg>"
  bus_selector11/21 -> outpmodule/462(VTPM_TPMSResButtAllow_flg)  "<VTPM_TPMSResButtAllow_flg>"
  bus_selector11/18 -> outpmodule/459(VTPM_LRWheelDebug_flg)  "<VTPM_LRWheelDebug_flg>"
  bus_selector11/17 -> outpmodule/458(VTPM_LFWheelDebug_flg)  "<VTPM_LFWheelDebug_flg>"
  bus_selector11/16 -> outpmodule/457(VTPM_RRSensorFail_flg)  "<VTPM_RRSensorFail_flg>"
  bus_selector11/15 -> outpmodule/456(VTPM_LRSensorFail_flg)  "<VTPM_LRSensorFail_flg>"
  bus_selector11/10 -> outpmodule/451(VTPM_RFWheelTemp_C)  "<VTPM_RFWheelTemp_C>"
  bus_selector11/9 -> outpmodule/450(VTPM_LFWheelTemp_C)  "<VTPM_LFWheelTemp_C>"
  bus_selector11/7 -> outpmodule/448(VTPM_LRWheelPress_raw8)  "<VTPM_LRWheelPress_raw8>"
  bus_selector11/8 -> outpmodule/449(VTPM_RRWheelPress_raw8)  "<VTPM_RRWheelPress_raw8>"
  bus_selector11/6 -> outpmodule/447(VTPM_RFWheelPress_raw8)  "<VTPM_RFWheelPress_raw8>"
  bus_selector11/39 -> outpmodule/480(VTPM_RFSensorMode_flg)  "<VTPM_RFSensorMode_flg>"
  bus_selector11/3 -> outpmodule/444(VTPM_LRBatWarn_flg)  "<VTPM_LRBatWarn_flg>"
  bus_selector11/4 -> outpmodule/445(VTPM_RRBatWarn_flg)  "<VTPM_RRBatWarn_flg>"
  bus_selector11/1 -> outpmodule/442(VTPM_LFBatWarn_flg)  "<VTPM_LFBatWarn_flg>"
  bus_selector11/26 -> outpmodule/467(VTPM_RRPressIndi_enum)  "<VTPM_RRPressIndi_enum>"
  bus_selector2/14 -> outpmodule/17(VAPM_APSDRLR_cm)  "<VAPM_APSDRLR_cm>"
  bus_selector2/2 -> outpmodule/5(VAPM_VehSpeedTimeOut_flg)  "<VAPM_VehSpeedTimeOut_flg>"
  bus_selector2/17 -> outpmodule/20(VAPM_APSDFLL_cm)  "<VAPM_APSDFLL_cm>"
  bus_selector2/9 -> outpmodule/12(VAPM_PASDRCL_cm)  "<VAPM_PASDRCL_cm>"
  bus_selector2/8 -> outpmodule/11(VAPM_PASDRCR_cm)  "<VAPM_PASDRCR_cm>"
  bus_selector2/7 -> outpmodule/10(VAPM_PASDRML_cm)  "<VAPM_PASDRML_cm>"
  bus_selector2/4 -> outpmodule/7(VAPM_FSOffSwTimeOut_flg)  "<VAPM_FSOffSwTimeOut_flg>"
  bus_selector2/3 -> outpmodule/6(VAPM_FSOffSw_enum)  "<VAPM_FSOffSw_enum>"
  bus_selector2/6 -> outpmodule/9(VAPM_PASDRMR_cm)  "<VAPM_PASDRMR_cm>"
  bus_selector2/28 -> outpmodule/31(VAPM_USSStaRLR_flg)  "<VAPM_USSStaRLR_flg>"
  bus_selector2/23 -> outpmodule/26(VAPM_PASAFMR_enum)  "<VAPM_PASAFMR_enum>"
  bus_selector15/44 -> outpmodule/628(VVMC_ADASVehSpdLim_raw32)  "<VVMC_ADASVehSpdLim_raw32>"
  bus_selector2/21 -> outpmodule/24(VAPM_PASARCR_enum)  "<VAPM_PASARCR_enum>"
  bus_selector2/18 -> outpmodule/21(VAPM_PASAFCL_enum)  "<VAPM_PASAFCL_enum>"
  bus_selector2/33 -> outpmodule/36(VAPM_USSStaFML_flg)  "<VAPM_USSStaFML_flg>"
  bus_selector2/19 -> outpmodule/22(VAPM_PASARMR_enum)  "<VAPM_PASARMR_enum>"
  BNMM_outputs/1 -> bus_selector7/1
  bus_selector7/11 -> outpmodule/304(VNMM_SysNMmSta_enum)  "<VNMM_SysNMmSta_enum>"
  bus_selector7/6 -> outpmodule/299(VNMM_NodeID_enum)  "<VNMM_NodeID_enum>"
  bus_selector7/7 -> outpmodule/300(VNMM_PNI_flg)  "<VNMM_PNI_flg>"
  bus_selector7/1 -> outpmodule/294(VNMM_AllCANTxReq_flg)  "<VNMM_AllCANTxReq_flg>"
  bus_selector7/4 -> outpmodule/297(VNMM_CSB_flg)  "<VNMM_CSB_flg>"
  bus_selector7/3 -> outpmodule/296(VNMM_Awake_enum)  "<VNMM_Awake_enum>"
  BDSC_outputs/1 -> bus_selector6/1
  bus_selector6/1 -> outpmodule/290(VDSC_DISCTurn_flg)  "<VDSC_DISCTurn_flg>"
  bus_selector10/11 -> outpmodule/400(VTHC_CoolgFanActDuty_pct)  "<VTHC_CoolgFanActDuty_pct>"
  bus_selector6/4 -> outpmodule/293(VDSC_DISCButtSta_flg)  "<VDSC_DISCButtSta_flg>"
  BDKC_outputs/1 -> bus_selector5/1
  bus_selector5/2 -> outpmodule/289(VDKC_DKCAuthSta_enum)  "<VDKC_DKCAuthSta_enum>"
  bus_selector5/1 -> outpmodule/288(VDKC_DKCTimeSN_cnt)  "<VDKC_DKCTimeSN_cnt>"
  BDHP_outputs/1 -> bus_selector4/1
  bus_selector4/1 -> outpmodule/285(VDHP_ActAPSPosn_pct)  "<VDHP_ActAPSPosn_pct>"
  BBCM_outputs/1 -> bus_selector3/1
  bus_selector3/119 -> outpmodule/284(VBCM_TurnSwSta_enum)  "<VBCM_TurnSwSta_enum>"
  bus_selector3/117 -> outpmodule/282(VBCM_FWipSwSta_enum)  "<VBCM_FWipSwSta_enum>"
  bus_selector3/116 -> outpmodule/281(VBCM_PassSWSta_flg)  "<VBCM_PassSWSta_flg>"
  bus_selector3/113 -> outpmodule/278(VBCM_AmbBrightnessSta7_enum)  "<VBCM_AmbBrightnessSta7_enum>"
  bus_selector3/115 -> outpmodule/280(VBCM_DimSwSta_flg)  "<VBCM_DimSwSta_flg>"
  bus_selector3/89 -> outpmodule/254(VBCM_AmbODAEN_flg)  "<VBCM_AmbODAEN_flg>"
  bus_selector3/90 -> outpmodule/255(VBCM_AmbColorSta_enum)  "<VBCM_AmbColorSta_enum>"
  bus_selector3/87 -> outpmodule/252(VBCM_AmbLinkDriSta_flg)  "<VBCM_AmbLinkDriSta_flg>"
  bus_selector3/88 -> outpmodule/253(VBCM_AmbPwrWarnEN_flg)  "<VBCM_AmbPwrWarnEN_flg>"
  bus_selector3/84 -> outpmodule/249(VBCM_AmbFunEN_flg)  "<VBCM_AmbFunEN_flg>"
  bus_selector3/83 -> outpmodule/248(VBCM_APMDoorControlSta_flg)  "<VBCM_APMDoorControlSta_flg>"
  bus_selector3/82 -> outpmodule/247(VBCM_LRRDCtrlCmd_pct)  "<VBCM_LRRDCtrlCmd_pct>"
  bus_selector3/80 -> outpmodule/245(VBCM_LPasCtrlCmd_pct)  "<VBCM_LPasCtrlCmd_pct>"
  bus_selector3/79 -> outpmodule/244(VBCM_LDrvCtrlCmd_pct)  "<VBCM_LDrvCtrlCmd_pct>"
  bus_selector3/81 -> outpmodule/246(VBCM_LRLDCtrlCmd_pct)  "<VBCM_LRLDCtrlCmd_pct>"
  bus_selector11/11 -> outpmodule/452(VTPM_LRWheelTemp_C)  "<VTPM_LRWheelTemp_C>"
  bus_selector3/77 -> outpmodule/242(VBCM_IVIPTGUSStaSW_flg)  "<VBCM_IVIPTGUSStaSW_flg>"
  bus_selector3/76 -> outpmodule/241(VBCM_RoomLampMode_flg)  "<VBCM_RoomLampMode_flg>"
  bus_selector3/73 -> outpmodule/238(VBCM_MirrorFlodPos_flg)  "<VBCM_MirrorFlodPos_flg>"
  bus_selector15/99 -> outpmodule/683(VVMC_VMCRWSActvSta_enum)  "<VVMC_VMCRWSActvSta_enum>"
  bus_selector3/72 -> outpmodule/237(VBCM_MFSWTri_flg)  "<VBCM_MFSWTri_flg>"
  bus_selector3/71 -> outpmodule/236(VBCM_CountAlarm_enum)  "<VBCM_CountAlarm_enum>"
  bus_selector3/69 -> outpmodule/234(VBCM_FollowMe_flg)  "<VBCM_FollowMe_flg>"
  bus_selector3/68 -> outpmodule/233(VBCM_APSOpenPTG_flg)  "<VBCM_APSOpenPTG_flg>"
  bus_selector3/70 -> outpmodule/235(VBCM_IVIRST_flg)  "<VBCM_IVIRST_flg>"
  bus_selector3/66 -> outpmodule/231(VBCM_LampPwr_flg)  "<VBCM_LampPwr_flg>"
  bus_selector3/65 -> outpmodule/230(VBCM_AmbLightColor6_enum)  "<VBCM_AmbLightColor6_enum>"
  bus_selector15/3 -> outpmodule/587(VVMC_VehicleSpeed_kph)  "<VVMC_VehicleSpeed_kph>"
  bus_selector3/62 -> outpmodule/227(VBCM_AmbLightColor3_enum)  "<VBCM_AmbLightColor3_enum>"
  bus_selector3/59 -> outpmodule/224(VBCM_AmbLightBrightness6_enum)  "<VBCM_AmbLightBrightness6_enum>"
  bus_selector3/61 -> outpmodule/226(VBCM_AmbLightColor2_enum)  "<VBCM_AmbLightColor2_enum>"
  bus_selector3/57 -> outpmodule/222(VBCM_AmbLightBrightness4_enum)  "<VBCM_AmbLightBrightness4_enum>"
  bus_selector3/55 -> outpmodule/220(VBCM_AmbLightBrightness2_enum)  "<VBCM_AmbLightBrightness2_enum>"
  bus_selector3/53 -> outpmodule/218(VBCM_AmbLightBreath6_enum)  "<VBCM_AmbLightBreath6_enum>"
  bus_selector3/54 -> outpmodule/219(VBCM_AmbLightBrightness1_enum)  "<VBCM_AmbLightBrightness1_enum>"
  bus_selector3/51 -> outpmodule/216(VBCM_AmbLightBreath4_enum)  "<VBCM_AmbLightBreath4_enum>"
  bus_selector3/52 -> outpmodule/217(VBCM_AmbLightBreath5_enum)  "<VBCM_AmbLightBreath5_enum>"
  bus_selector3/50 -> outpmodule/215(VBCM_AmbLightBreath3_enum)  "<VBCM_AmbLightBreath3_enum>"
  bus_selector3/49 -> outpmodule/214(VBCM_AmbLightBreath2_enum)  "<VBCM_AmbLightBreath2_enum>"
  bus_selector3/48 -> outpmodule/213(VBCM_AmbLightBreath1_enum)  "<VBCM_AmbLightBreath1_enum>"
  bus_selector3/45 -> outpmodule/210(VBCM_RrWiper_flg)  "<VBCM_RrWiper_flg>"
  bus_selector3/109 -> outpmodule/274(VBCM_AmbBrightnessSta2_enum)  "<VBCM_AmbBrightnessSta2_enum>"
  bus_selector3/43 -> outpmodule/208(VBCM_FrWiperL_flg)  "<VBCM_FrWiperL_flg>"
  bus_selector11/12 -> outpmodule/453(VTPM_RRWheelTemp_C)  "<VTPM_RRWheelTemp_C>"
  bus_selector3/36 -> outpmodule/201(VBCM_MirrorCtrl_enum)  "<VBCM_MirrorCtrl_enum>"
  bus_selector3/38 -> outpmodule/203(VBCM_RrDefog_flg)  "<VBCM_RrDefog_flg>"
  bus_selector3/37 -> outpmodule/202(VBCM_MirrorDefog_flg)  "<VBCM_MirrorDefog_flg>"
  bus_selector3/34 -> outpmodule/199(VBCM_RTurnLP_flg)  "<VBCM_RTurnLP_flg>"
  bus_selector3/33 -> outpmodule/198(VBCM_LTurnLP_flg)  "<VBCM_LTurnLP_flg>"
  bus_selector3/32 -> outpmodule/197(VBCM_HazardSW_flg)  "<VBCM_HazardSW_flg>"
  bus_selector3/29 -> outpmodule/194(VBCM_RDRL_flg)  "<VBCM_RDRL_flg>"
  bus_selector3/25 -> outpmodule/190(VBCM_RrFogLamp_flg)  "<VBCM_RrFogLamp_flg>"
  bus_selector3/28 -> outpmodule/193(VBCM_LDRL_flg)  "<VBCM_LDRL_flg>"
  bus_selector3/26 -> outpmodule/191(VBCM_BrakeLamp_flg)  "<VBCM_BrakeLamp_flg>"
  bus_selector3/24 -> outpmodule/189(VBCM_HBeam_flg)  "<VBCM_HBeam_flg>"
  bus_selector3/21 -> outpmodule/186(VBCM_DimmerEN_flg)  "<VBCM_DimmerEN_flg>"
  bus_selector3/19 -> outpmodule/184(VBCM_CTDLockSW_flg)  "<VBCM_CTDLockSW_flg>"
  bus_selector3/20 -> outpmodule/185(VBCM_Dimmer_pct)  "<VBCM_Dimmer_pct>"
  bus_selector3/22 -> outpmodule/187(VBCM_PosLamp_flg)  "<VBCM_PosLamp_flg>"
  bus_selector3/16 -> outpmodule/181(VBCM_CrashDetd_flg)  "<VBCM_CrashDetd_flg>"
  bus_selector3/18 -> outpmodule/183(VBCM_DoorLockIND_flg)  "<VBCM_DoorLockIND_flg>"
  bus_selector3/15 -> outpmodule/180(VBCM_RrChargingDoorCtrl_enum)  "<VBCM_RrChargingDoorCtrl_enum>"
  bus_selector10/38 -> outpmodule/427(VTHC_ACSubMode_enum)  "<VTHC_ACSubMode_enum>"
  bus_selector3/9 -> outpmodule/174(VBCM_DrDoorSW_flg)  "<VBCM_DrDoorSW_flg>"
  bus_selector3/10 -> outpmodule/175(VBCM_PsDoorSW_flg)  "<VBCM_PsDoorSW_flg>"
  bus_selector2/10 -> outpmodule/13(VAPM_PASDFMR_cm)  "<VAPM_PASDFMR_cm>"
  bus_selector3/12 -> outpmodule/177(VBCM_RRDoorSW_flg)  "<VBCM_RRDoorSW_flg>"
  bus_selector3/7 -> outpmodule/172(VBCM_HoodSW_flg)  "<VBCM_HoodSW_flg>"
  bus_selector3/5 -> outpmodule/170(VBCM_BCMDoorLockSta_flg)  "<VBCM_BCMDoorLockSta_flg>"
  bus_selector2/55 -> outpmodule/58(VAPM_RFRawWhlSpeedVTimeOut_flg)  "<VAPM_RFRawWhlSpeedVTimeOut_flg>"
  bus_selector2/54 -> outpmodule/57(VAPM_RFRawWhlSpeedV_flg)  "<VAPM_RFRawWhlSpeedV_flg>"
  bus_selector10/9 -> outpmodule/398(VTHC_FDTWVCmd_pct)  "<VTHC_FDTWVCmd_pct>"
  bus_selector2/73 -> outpmodule/76(VAPM_LRPulseCountVTimeOut_flg)  "<VAPM_LRPulseCountVTimeOut_flg>"
  bus_selector10/2 -> outpmodule/391(VTHC_FDSOV1Cmd_flg)  "<VTHC_FDSOV1Cmd_flg>"
  bus_selector2/53 -> outpmodule/56(VAPM_LFRawWhlSpeedVTimeOut_flg)  "<VAPM_LFRawWhlSpeedVTimeOut_flg>"
  bus_selector2/51 -> outpmodule/54(VAPM_RRRawWhlSpeedTimeOut_flg)  "<VAPM_RRRawWhlSpeedTimeOut_flg>"
  bus_selector2/69 -> outpmodule/72(VAPM_LFPulseCountVTimeOut_flg)  "<VAPM_LFPulseCountVTimeOut_flg>"
  bus_selector2/66 -> outpmodule/69(VAPM_RRWhlRotDir_enum)  "<VAPM_RRWhlRotDir_enum>"
  bus_selector2/62 -> outpmodule/65(VAPM_RFWhlRotDir_enum)  "<VAPM_RFWhlRotDir_enum>"
  bus_selector2/59 -> outpmodule/62(VAPM_RRRawWhlSpeedVTimeOut_flg)  "<VAPM_RRRawWhlSpeedVTimeOut_flg>"
  bus_selector1/2 -> outpmodule/2(VACC_LVBattVoltSta_enum)  "<VACC_LVBattVoltSta_enum>"
  bus_selector2/12 -> outpmodule/15(VAPM_PASDFCR_cm)  "<VAPM_PASDFCR_cm>"
  bus_selector2/16 -> outpmodule/19(VAPM_APSDFLR_cm)  "<VAPM_APSDFLR_cm>"
  bus_selector8/8 -> outpmodule/313(VPMM_HVBatCnctReq_flg)  "<VPMM_HVBatCnctReq_flg>"
  bus_selector8/4 -> outpmodule/309(VPMM_PowerDownFault_enum)  "<VPMM_PowerDownFault_enum>"
  bus_selector8/3 -> outpmodule/308(VPMM_PowerUpFault_enum)  "<VPMM_PowerUpFault_enum>"
  BSYS_outputs/1 -> bus_selector9/1
  bus_selector8/12 -> outpmodule/317(VPMM_HVPwrSta_flg)  "<VPMM_HVPwrSta_flg>"
  bus_selector2/124 -> outpmodule/127(VAPM_ESCAPSSta_enum)  "<VAPM_ESCAPSSta_enum>"
  bus_selector2/106 -> outpmodule/109(VAPM_LongAccel_Gps)  "<VAPM_LongAccel_Gps>"
  bus_selector2/125 -> outpmodule/128(VAPM_ESCAPSStaTimeOut_flg)  "<VAPM_ESCAPSStaTimeOut_flg>"
  bus_selector2/122 -> outpmodule/125(VAPM_ESCStandstill_flg)  "<VAPM_ESCStandstill_flg>"
  bus_selector2/117 -> outpmodule/120(VAPM_MCPressureVTimeOut_flg)  "<VAPM_MCPressureVTimeOut_flg>"
  bus_selector2/116 -> outpmodule/119(VAPM_MCPressureV_bar)  "<VAPM_MCPressureV_bar>"
  bus_selector2/20 -> outpmodule/23(VAPM_PASARML_enum)  "<VAPM_PASARML_enum>"
  bus_selector2/113 -> outpmodule/116(VAPM_LatAccelVTimeOut_flg)  "<VAPM_LatAccelVTimeOut_flg>"
  bus_selector8/14 -> outpmodule/319(VPMM_FrMCUEnaReq_flg)  "<VPMM_FrMCUEnaReq_flg>"
  bus_selector2/112 -> outpmodule/115(VAPM_LatAccelV_flg)  "<VAPM_LatAccelV_flg>"
  bus_selector8/18 -> outpmodule/323(VPMM_PwrStaSelect_enum)  "<VPMM_PwrStaSelect_enum>"
  bus_selector9/32 -> outpmodule/385(VSYS_FdcSlpTime_sec)  "<VSYS_FdcSlpTime_sec>"
  bus_selector9/29 -> outpmodule/382(VSYS_SHA8_cnt)  "<VSYS_SHA8_cnt>"
  bus_selector11/5 -> outpmodule/446(VTPM_LFWheelPress_raw8)  "<VTPM_LFWheelPress_raw8>"
  bus_selector3/110 -> outpmodule/275(VBCM_AmbBrightnessSta3_enum)  "<VBCM_AmbBrightnessSta3_enum>"
  bus_selector3/107 -> outpmodule/272(VBCM_AmbColorSta7_enum)  "<VBCM_AmbColorSta7_enum>"
  outpmodule/341(VOUTP_LVSilentChrgReq_flg) -> bus_creator/341
  bus_selector3/112 -> outpmodule/277(VBCM_AmbBrightnessSta5_enum)  "<VBCM_AmbBrightnessSta5_enum>"
  bus_selector3/101 -> outpmodule/266(VBCM_AmbODAENFlash_enum)  "<VBCM_AmbODAENFlash_enum>"
  bus_selector3/99 -> outpmodule/264(VBCM_AmbLinkDriStaFlash_enum)  "<VBCM_AmbLinkDriStaFlash_enum>"
  bus_selector10/14 -> outpmodule/403(VTHC_FDEWP2Cmd_enum)  "<VTHC_FDEWP2Cmd_enum>"
  bus_selector3/111 -> outpmodule/276(VBCM_AmbBrightnessSta4_enum)  "<VBCM_AmbBrightnessSta4_enum>"
  bus_selector15/38 -> outpmodule/622(VVMC_ACCObjRelSpd_mps)  "<VVMC_ACCObjRelSpd_mps>"
  BAPM_outputs/1 -> bus_selector2/1
  bus_selector2/161 -> outpmodule/164(VAPM_APSRqEPASCtrl_flg)  "<VAPM_APSRqEPASCtrl_flg>"
  outpmodule/88(VOUTP_ShifterHandleCmdTimeOut_flg) -> bus_creator/88
  bus_selector2/159 -> outpmodule/162(VAPM_APSAngleTarget_Deg)  "<VAPM_APSAngleTarget_Deg>"
  bus_selector2/160 -> outpmodule/163(VAPM_APSVRqEPASCtrl_flg)  "<VAPM_APSVRqEPASCtrl_flg>"
  bus_selector11/45 -> outpmodule/486(VTPM_S4ID_raw32)  "<VTPM_S4ID_raw32>"
  bus_selector8/5 -> outpmodule/310(VPMM_ActiveDischargeReq_flg)  "<VPMM_ActiveDischargeReq_flg>"
  bus_selector2/156 -> outpmodule/159(VAPM_APSSWVer_enum)  "<VAPM_APSSWVer_enum>"
  bus_selector8/17 -> outpmodule/322(VPMM_DrSeatSta_enum)  "<VPMM_DrSeatSta_enum>"
  bus_selector2/158 -> outpmodule/161(VAPM_APSExitCondition_enum)  "<VAPM_APSExitCondition_enum>"
  bus_selector2/153 -> outpmodule/156(VAPM_DriverSeatBeltCmdTimeOut_flg)  "<VAPM_DriverSeatBeltCmdTimeOut_flg>"
  bus_selector2/150 -> outpmodule/153(VAPM_TCSActive_flg)  "<VAPM_TCSActive_flg>"
  bus_selector2/151 -> outpmodule/154(VAPM_TCSActiveTimeOut_flg)  "<VAPM_TCSActiveTimeOut_flg>"
  outpmodule/89(VOUTP_DriIntend_enum) -> bus_creator/89
  bus_selector2/149 -> outpmodule/152(VAPM_ABSActiveTimeOut_flg)  "<VAPM_ABSActiveTimeOut_flg>"
  bus_selector2/5 -> outpmodule/8(VAPM_ChrgPlugSta_enum)  "<VAPM_ChrgPlugSta_enum>"
  bus_selector2/141 -> outpmodule/144(VAPM_AVMErrSTATimeOut_flg)  "<VAPM_AVMErrSTATimeOut_flg>"
  bus_selector2/139 -> outpmodule/142(VAPM_AVMParkingmodeTimeOut_flg)  "<VAPM_AVMParkingmodeTimeOut_flg>"
  bus_selector15/91 -> outpmodule/675(VVMC_APSStaSys_enum)  "<VVMC_APSStaSys_enum>"
  bus_selector2/137 -> outpmodule/140(VAPM_AVMparkingexcuteTimeOut_flg)  "<VAPM_AVMparkingexcuteTimeOut_flg>"
  bus_selector2/133 -> outpmodule/136(VAPM_EPBStaTimeOut_flg)  "<VAPM_EPBStaTimeOut_flg>"
  bus_selector2/131 -> outpmodule/134(VAPM_EPBErrStaTimeOut_flg)  "<VAPM_EPBErrStaTimeOut_flg>"
  bus_selector3/108 -> outpmodule/273(VBCM_AmbBrightnessSta1_enum)  "<VBCM_AmbBrightnessSta1_enum>"
  bus_selector2/134 -> outpmodule/137(VAPM_AVMparkingcancel_enum)  "<VAPM_AVMparkingcancel_enum>"
  bus_selector10/29 -> outpmodule/418(VTHC_sigRecircSt_flg)  "<VTHC_sigRecircSt_flg>"
  bus_creator/1 -> BOUTP_outputs/1
  bus_selector2/130 -> outpmodule/133(VAPM_EPBErrSta_enum)  "<VAPM_EPBErrSta_enum>"
  bus_selector2/44 -> outpmodule/47(VAPM_LFRawWhlSpeed_kph)  "<VAPM_LFRawWhlSpeed_kph>"
  bus_selector2/43 -> outpmodule/46(VAPM_BrkPedalPosTimeOut_flg)  "<VAPM_BrkPedalPosTimeOut_flg>"
  bus_selector2/70 -> outpmodule/73(VAPM_RFPulseCountV_flg)  "<VAPM_RFPulseCountV_flg>"
  bus_selector11/19 -> outpmodule/460(VTPM_RFWheelDebug_flg)  "<VTPM_RFWheelDebug_flg>"
  bus_selector2/42 -> outpmodule/45(VAPM_BrkPedalPos_pct)  "<VAPM_BrkPedalPos_pct>"
  outpmodule/615(VOUTP_ADASAEBReq_enum) -> bus_creator/615
  outpmodule/620(VOUTP_ADASACCSta_enum) -> bus_creator/620
  bus_selector15/64 -> outpmodule/648(VVMC_ADASLaneModeL_enum)  "<VVMC_ADASLaneModeL_enum>"
  outpmodule/613(VOUTP_LKATOIFault_flg) -> bus_creator/613
  outpmodule/610(VOUTP_LateralCtrl_flg) -> bus_creator/610
  bus_selector15/62 -> outpmodule/646(VVMC_LKAHODSoundWarning_flg)  "<VVMC_LKAHODSoundWarning_flg>"
  bus_selector11/43 -> outpmodule/484(VTPM_S2ID_raw32)  "<VTPM_S2ID_raw32>"
  bus_selector3/97 -> outpmodule/262(VBCM_AmbWelENFlash_enum)  "<VBCM_AmbWelENFlash_enum>"
  outpmodule/609(VOUTP_FeatArbitrFinal_enum) -> bus_creator/609
  outpmodule/621(VOUTP_ACCObjDist_m) -> bus_creator/621
  bus_selector11/42 -> outpmodule/483(VTPM_S1ID_raw32)  "<VTPM_S1ID_raw32>"
  outpmodule/602(VOUTP_SPD2ACCAct_flg) -> bus_creator/602
  outpmodule/600(VOUTP_LatAccCtrl_flg) -> bus_creator/600
  outpmodule/596(VOUTP_LimitPCT_pct) -> bus_creator/596
  bus_selector2/127 -> outpmodule/130(VAPM_EPBExtReleaseAvailTimeOut_flg)  "<VAPM_EPBExtReleaseAvailTimeOut_flg>"
  outpmodule/592(VOUTP_VMCMSACtrlAvail_flg) -> bus_creator/592
  outpmodule/593(VOUTP_FeatArbitrSta_enum) -> bus_creator/593
  outpmodule/619(VOUTP_ADASDBSReq_enum) -> bus_creator/619
  outpmodule/580(VOUTP_SetSpd_kph) -> bus_creator/580
  outpmodule/618(VOUTP_ACCVehHoldReq_flg) -> bus_creator/618
  outpmodule/574(VOUTP_IVIPwrLockSta_enum) -> bus_creator/574
  bus_selector8/6 -> outpmodule/311(VPMM_DCDCEnaReq_flg)  "<VPMM_DCDCEnaReq_flg>"
  outpmodule/571(VOUTP_EquivAccPedalSWSta_flg) -> bus_creator/571
  bus_selector10/41 -> outpmodule/430(VTHC_Face_flg)  "<VTHC_Face_flg>"
  outpmodule/570(VOUTP_CreepON_flg) -> bus_creator/570
  outpmodule/568(VOUTP_RrUdcMax_V) -> bus_creator/568
  outpmodule/606(VOUTP_ISOJerkLimit_mps3) -> bus_creator/606
  outpmodule/569(VOUTP_ReBrakeLPReq_flg) -> bus_creator/569
  outpmodule/566(VOUTP_RrIdcMax_A) -> bus_creator/566
  bus_selector8/20 -> outpmodule/325(VPMM_TCountSta_enum)  "<VPMM_TCountSta_enum>"
  outpmodule/565(VOUTP_RrIdcMin_A) -> bus_creator/565
  outpmodule/564(VOUTP_FrUdcMax_V) -> bus_creator/564
  outpmodule/563(VOUTP_FrUdcMin_V) -> bus_creator/563
  bus_selector3/3 -> outpmodule/168(VBCM_HornCtrl_flg)  "<VBCM_HornCtrl_flg>"
  outpmodule/579(VOUTP_SpdCtrlSta_flg) -> bus_creator/579
  outpmodule/562(VOUTP_FrIdcMax_A) -> bus_creator/562
  outpmodule/558(VOUTP_PTCSPermSta_flg) -> bus_creator/558
  outpmodule/598(VOUTP_RearWhlSlipRatioCtrl_flg) -> bus_creator/598
  bus_selector3/35 -> outpmodule/200(VBCM_BCMBuzzerReq_flg)  "<VBCM_BCMBuzzerReq_flg>"
  outpmodule/556(VOUTP_RrEDUAvailBrkRgnTqV_flg) -> bus_creator/556
  bus_selector3/106 -> outpmodule/271(VBCM_AmbColorSta5_enum)  "<VBCM_AmbColorSta5_enum>"
  outpmodule/552(VOUTP_RrEDUSpd_rpm) -> bus_creator/552
  bus_selector7/10 -> outpmodule/303(VNMM_ActiveWU_flg)  "<VNMM_ActiveWU_flg>"
  outpmodule/549(VOUTP_FrEDURolRgnTq_Nm) -> bus_creator/549
  outpmodule/547(VOUTP_FrEDUActTq_Nm) -> bus_creator/547
  outpmodule/544(VOUTP_RrRgnDecrSta_flg) -> bus_creator/544
  outpmodule/585(VOUTP_FeatSetSpdFinal_raw32) -> bus_creator/585
  outpmodule/545(VOUTP_DriverWhlTqDemFr_Nm) -> bus_creator/545
  outpmodule/539(VOUTP_ShiftGearPosn_enum) -> bus_creator/539
  outpmodule/532(VOUTP_FlashIDvalid_enum) -> bus_creator/532
  outpmodule/531(VOUTP_FlashS4ID_raw) -> bus_creator/531
  outpmodule/527(VOUTP_Prepresstempvalid_enum) -> bus_creator/527
  outpmodule/525(VOUTP_unlearnSfali_flg) -> bus_creator/525
  outpmodule/522(VOUTP_WriteChkfinRRID_raw) -> bus_creator/522
  outpmodule/521(VOUTP_WriteChkfinLRID_raw) -> bus_creator/521
  outpmodule/611(VOUTP_ADASLKASta_enum) -> bus_creator/611
  bus_selector8/15 -> outpmodule/320(VPMM_RrMCUEnaReq_flg)  "<VPMM_RrMCUEnaReq_flg>"
  outpmodule/518(VOUTP_WriteChkRRID_raw) -> bus_creator/518
  outpmodule/519(VOUTP_WriteChkfinLFID_raw) -> bus_creator/519
  bus_selector2/157 -> outpmodule/160(VAPM_APSHWVer_enum)  "<VAPM_APSHWVer_enum>"
  outpmodule/515(VOUTP_WriteChkLFID_raw) -> bus_creator/515
  outpmodule/587(VOUTP_VehicleSpeed_kph) -> bus_creator/587
  outpmodule/512(VOUTP_RFPind_enum) -> bus_creator/512
  outpmodule/508(VOUTP_TPMSStorge_flg) -> bus_creator/508
  outpmodule/509(VOUTP_ChkStorge_flg) -> bus_creator/509
  outpmodule/505(VOUTP_ID4messageALTU_raw8) -> bus_creator/505
  outpmodule/506(VOUTP_Chkfin_flg) -> bus_creator/506
  outpmodule/504(VOUTP_ID3messageALTU_raw8) -> bus_creator/504
  outpmodule/501(VOUTP_S4WheelDebugALTU_pct) -> bus_creator/501
  outpmodule/575(VOUTP_OPDHoldLamp_flg) -> bus_creator/575
  outpmodule/542(VOUTP_RrActvDmpDisabReq_flg) -> bus_creator/542
  outpmodule/494(VOUTP_LRP20_raw8) -> bus_creator/494
  outpmodule/491(VOUTP_ALFin_flg) -> bus_creator/491
  outpmodule/488(VOUTP_S2L_enum) -> bus_creator/488
  bus_selector9/30 -> outpmodule/383(VSYS_NvWriteReqRisingEdge_flg)  "<VSYS_NvWriteReqRisingEdge_flg>"
  outpmodule/486(VOUTP_S4ID_raw32) -> bus_creator/486
  outpmodule/487(VOUTP_S1L_enum) -> bus_creator/487
  outpmodule/484(VOUTP_S2ID_raw32) -> bus_creator/484
  outpmodule/481(VOUTP_LRSensorMode_flg) -> bus_creator/481
  outpmodule/548(VOUTP_RrEDUActTq_Nm) -> bus_creator/548
  outpmodule/479(VOUTP_LFSensorMode_flg) -> bus_creator/479
  outpmodule/478(VOUTP_AutoLTips_enum) -> bus_creator/478
  outpmodule/477(VOUTP_CWheelTips_enum) -> bus_creator/477
  outpmodule/476(VOUTP_RRWheelPSW_raw8) -> bus_creator/476
  outpmodule/475(VOUTP_RFWheelPSW_raw8) -> bus_creator/475
  outpmodule/473(VOUTP_LFWheelPSW_raw8) -> bus_creator/473
  outpmodule/524(VOUTP_Flashdatavalid_enum) -> bus_creator/524
  outpmodule/471(VOUTP_LRWheelTmpIndi_flg) -> bus_creator/471
  outpmodule/465(VOUTP_RFPressIndi_enum) -> bus_creator/465
  outpmodule/451(VOUTP_RFWheelTemp_C) -> bus_creator/451
  outpmodule/452(VOUTP_LRWheelTemp_C) -> bus_creator/452
  outpmodule/498(VOUTP_S1WheelDebugALTU_pct) -> bus_creator/498
  outpmodule/591(VOUTP_VMCCCCtrlAvail_flg) -> bus_creator/591
  outpmodule/448(VOUTP_LRWheelPress_raw8) -> bus_creator/448
  outpmodule/449(VOUTP_RRWheelPress_raw8) -> bus_creator/449
  outpmodule/447(VOUTP_RFWheelPress_raw8) -> bus_creator/447
  outpmodule/445(VOUTP_RRBatWarn_flg) -> bus_creator/445
  outpmodule/441(VOUTP_FDCTHCMAPTCWarningSta_flg) -> bus_creator/441
  bus_selector15/45 -> outpmodule/629(VVMC_ADASShftPosnReqA_flg)  "<VVMC_ADASShftPosnReqA_flg>"
  bus_selector3/96 -> outpmodule/261(VBCM_AmbFunENFlash_enum)  "<VBCM_AmbFunENFlash_enum>"
  outpmodule/442(VOUTP_LFBatWarn_flg) -> bus_creator/442
  outpmodule/440(VOUTP_sigSetTempZon2StM_C) -> bus_creator/440
  outpmodule/434(VOUTP_FootM_flg) -> bus_creator/434
  outpmodule/432(VOUTP_Frost_flg) -> bus_creator/432
  outpmodule/431(VOUTP_Foot_flg) -> bus_creator/431
  outpmodule/425(VOUTP_sigAmbAirT_C) -> bus_creator/425
  bus_selector8/16 -> outpmodule/321(VPMM_DrivetrainSelect_enum)  "<VPMM_DrivetrainSelect_enum>"
  outpmodule/423(VOUTP_sigClntTHvBattIn_C) -> bus_creator/423
  outpmodule/500(VOUTP_S3WheelDebugALTU_pct) -> bus_creator/500
  outpmodule/396(VOUTP_FDSOTXVCmd_flg) -> bus_creator/396
  bus_selector15/36 -> outpmodule/620(VVMC_ADASACCSta_enum)  "<VVMC_ADASACCSta_enum>"
  outpmodule/395(VOUTP_FDEXV2Cmd_step) -> bus_creator/395
  outpmodule/394(VOUTP_FDEXV1Cmd_step) -> bus_creator/394
  outpmodule/482(VOUTP_RRSensorMode_flg) -> bus_creator/482
  outpmodule/430(VOUTP_Face_flg) -> bus_creator/430
  outpmodule/389(VOUTP_CurrentNmState_enum) -> bus_creator/389
  outpmodule/390(VOUTP_FDCompCmd_rpm) -> bus_creator/390
  outpmodule/94(VOUTP_SASAngleTimeOut_flg) -> bus_creator/94
  outpmodule/387(VOUTP_WisrBootReason_raw32) -> bus_creator/387
  bus_selector2/136 -> outpmodule/139(VAPM_AVMparkingexcute_enum)  "<VAPM_AVMparkingexcute_enum>"
  outpmodule/385(VOUTP_FdcSlpTime_sec) -> bus_creator/385
  outpmodule/386(VOUTP_PmicBootReason_enum) -> bus_creator/386
  bus_selector2/107 -> outpmodule/110(VAPM_LongAccelTimeOut_flg)  "<VAPM_LongAccelTimeOut_flg>"
  outpmodule/383(VOUTP_NvWriteReqRisingEdge_flg) -> bus_creator/383
  bus_selector15/57 -> outpmodule/641(VVMC_ADASWarningMsg_enum)  "<VVMC_ADASWarningMsg_enum>"
  bus_selector15/61 -> outpmodule/645(VVMC_LKAHODDisplayWarning_flg)  "<VVMC_LKAHODDisplayWarning_flg>"
  outpmodule/458(VOUTP_LFWheelDebug_flg) -> bus_creator/458
  outpmodule/384(VOUTP_FdcSlpReqRisingEdge_flg) -> bus_creator/384
  bus_selector15/82 -> outpmodule/666(VVMC_ADASAEBSta_enum)  "<VVMC_ADASAEBSta_enum>"
  outpmodule/573(VOUTP_ActParkRequest_flg) -> bus_creator/573
  outpmodule/382(VOUTP_SHA8_cnt) -> bus_creator/382
  outpmodule/381(VOUTP_SHA7_cnt) -> bus_creator/381
  outpmodule/414(VOUTP_CCUACMaxLampSts_flg) -> bus_creator/414
  outpmodule/413(VOUTP_CCUAutoLampSts_flg) -> bus_creator/413
  bus_selector8/11 -> outpmodule/316(VPMM_LVPwrSta_flg)  "<VPMM_LVPwrSta_flg>"
  bus_selector2/108 -> outpmodule/111(VAPM_MCPressure_bar)  "<VAPM_MCPressure_bar>"
  outpmodule/409(VOUTP_BatteryMode_enum) -> bus_creator/409
  outpmodule/411(VOUTP_CabinMode_enum) -> bus_creator/411
  outpmodule/407(VOUTP_FDRrAPTCHeatPwrCmd_W) -> bus_creator/407
  outpmodule/404(VOUTP_FDEWP3Cmd_enum) -> bus_creator/404
  bus_selector3/14 -> outpmodule/179(VBCM_FrChargingDoorCtrl_enum)  "<VBCM_FrChargingDoorCtrl_enum>"
  outpmodule/402(VOUTP_FDEWP1Cmd_enum) -> bus_creator/402
  bus_selector2/115 -> outpmodule/118(VAPM_LongAccelVTimeOut_flg)  "<VAPM_LongAccelVTimeOut_flg>"
  outpmodule/401(VOUTP_FDAGSCmd_enum) -> bus_creator/401
  outpmodule/399(VOUTP_FDFrWPTCHeatPwrCmd_W) -> bus_creator/399
  outpmodule/333(VOUTP_IVIPwrStaONTOPopT_s) -> bus_creator/333
  bus_selector2/162 -> outpmodule/165(VAPM_CAASSta_enum)  "<VAPM_CAASSta_enum>"
  outpmodule/331(VOUTP_EvccAplusPwrUpReq_flg) -> bus_creator/331
  outpmodule/420(VOUTP_sigSetTempZon2St_C) -> bus_creator/420
  outpmodule/324(VOUTP_PwrStaConstraint_enum) -> bus_creator/324
  outpmodule/513(VOUTP_LRPindi_enum) -> bus_creator/513
  outpmodule/322(VOUTP_DrSeatSta_enum) -> bus_creator/322
  outpmodule/321(VOUTP_DrivetrainSelect_enum) -> bus_creator/321
  outpmodule/318(VOUTP_SysPowerMode_enum) -> bus_creator/318
  bus_selector2/22 -> outpmodule/25(VAPM_PASARCL_enum)  "<VAPM_PASARCL_enum>"
  outpmodule/510(VOUTP_TPMSResButt_flg) -> bus_creator/510
  outpmodule/319(VOUTP_FrMCUEnaReq_flg) -> bus_creator/319
  outpmodule/422(VOUTP_sigCbnSolarLeft_W) -> bus_creator/422
  bus_selector8/22 -> outpmodule/327(VPMM_PwrDownReq_enum)  "<VPMM_PwrDownReq_enum>"
  outpmodule/320(VOUTP_RrMCUEnaReq_flg) -> bus_creator/320
  bus_selector15/31 -> outpmodule/615(VVMC_ADASAEBReq_enum)  "<VVMC_ADASAEBReq_enum>"
  outpmodule/317(VOUTP_HVPwrSta_flg) -> bus_creator/317
  outpmodule/511(VOUTP_LFPindi_enum) -> bus_creator/511
  outpmodule/316(VOUTP_LVPwrSta_flg) -> bus_creator/316
  outpmodule/314(VOUTP_HVSysReadyToCharge_enum) -> bus_creator/314
  bus_selector3/78 -> outpmodule/243(VBCM_PTGInnerSW2_enum)  "<VBCM_PTGInnerSW2_enum>"
  outpmodule/419(VOUTP_sigSetTempZon1St_C) -> bus_creator/419
  outpmodule/601(VOUTP_SafetyCtrl_flg) -> bus_creator/601
  outpmodule/313(VOUTP_HVBatCnctReq_flg) -> bus_creator/313
  outpmodule/312(VOUTP_DCDCVoltSetpoint_V) -> bus_creator/312
  outpmodule/309(VOUTP_PowerDownFault_enum) -> bus_creator/309
  bus_selector2/46 -> outpmodule/49(VAPM_RFRawWhlSpeed_kph)  "<VAPM_RFRawWhlSpeed_kph>"
  outpmodule/546(VOUTP_DriverWhlTqDemRr_Nm) -> bus_creator/546
  outpmodule/311(VOUTP_DCDCEnaReq_flg) -> bus_creator/311
  outpmodule/308(VOUTP_PowerUpFault_enum) -> bus_creator/308
  outpmodule/307(VOUTP_PowerDownState_enum) -> bus_creator/307
  bus_selector3/27 -> outpmodule/192(VBCM_ReverseLamp_flg)  "<VBCM_ReverseLamp_flg>"
  bus_selector2/49 -> outpmodule/52(VAPM_LRRawWhlSpeedTimeOut_flg)  "<VAPM_LRRawWhlSpeedTimeOut_flg>"
  outpmodule/480(VOUTP_RFSensorMode_flg) -> bus_creator/480
  outpmodule/305(VOUTP_NetworkReq_flg) -> bus_creator/305
  outpmodule/340(VOUTP_LVSilentChrgSta_enum) -> bus_creator/340
  outpmodule/302(VOUTP_WakeUp_enum) -> bus_creator/302
  outpmodule/304(VOUTP_SysNMmSta_enum) -> bus_creator/304
  outpmodule/393(VOUTP_FDSOV3Cmd_flg) -> bus_creator/393
  outpmodule/424(VOUTP_sigCbnSolarRight_W) -> bus_creator/424
  outpmodule/303(VOUTP_ActiveWU_flg) -> bus_creator/303
  outpmodule/301(VOUTP_RptMsgReq_flg) -> bus_creator/301
  outpmodule/300(VOUTP_PNI_flg) -> bus_creator/300
  outpmodule/299(VOUTP_NodeID_enum) -> bus_creator/299
  bus_selector15/58 -> outpmodule/642(VVMC_ADASCAMSpdLim_enum)  "<VVMC_ADASCAMSpdLim_enum>"
  outpmodule/298(VOUTP_ErrorState_enum) -> bus_creator/298
  outpmodule/577(VOUTP_FDCVCURegenMode_enum) -> bus_creator/577
  outpmodule/296(VOUTP_Awake_enum) -> bus_creator/296
  bus_selector15/28 -> outpmodule/612(VVMC_LKAStrToqReq_Nm)  "<VVMC_LKAStrToqReq_Nm>"
  outpmodule/294(VOUTP_AllCANTxReq_flg) -> bus_creator/294
  outpmodule/293(VOUTP_DISCButtSta_flg) -> bus_creator/293
  bus_selector3/1 -> outpmodule/166(VBCM_AntitheftSta_enum)  "<VBCM_AntitheftSta_enum>"
  outpmodule/292(VOUTP_DISCSta_enum) -> bus_creator/292
  outpmodule/612(VOUTP_LKAStrToqReq_Nm) -> bus_creator/612
  outpmodule/290(VOUTP_DISCTurn_flg) -> bus_creator/290
  outpmodule/288(VOUTP_DKCTimeSN_cnt) -> bus_creator/288
  outpmodule/289(VOUTP_DKCAuthSta_enum) -> bus_creator/289
  outpmodule/586(VOUTP_VehicleSpeed_mph) -> bus_creator/586
  outpmodule/287(VOUTP_EAPS2MIN_pct) -> bus_creator/287
  outpmodule/286(VOUTP_EAPS1MIN_pct) -> bus_creator/286
  outpmodule/284(VOUTP_TurnSwSta_enum) -> bus_creator/284
  outpmodule/283(VOUTP_FWasSwSta_enum) -> bus_creator/283
  outpmodule/281(VOUTP_PassSWSta_flg) -> bus_creator/281
  outpmodule/282(VOUTP_FWipSwSta_enum) -> bus_creator/282
  outpmodule/406(VOUTP_FDFrRiAPTCHeatPwrCmd_W) -> bus_creator/406
  outpmodule/279(VOUTP_HazardIND_flg) -> bus_creator/279
  outpmodule/604(VOUTP_ISOAccLimit_mps2) -> bus_creator/604
  outpmodule/416(VOUTP_sigAirIntenZon1St_enum) -> bus_creator/416
  outpmodule/418(VOUTP_sigRecircSt_flg) -> bus_creator/418
  outpmodule/417(VOUTP_sigWindDirZon1St_enum) -> bus_creator/417
  outpmodule/271(VOUTP_AmbColorSta5_enum) -> bus_creator/271
  outpmodule/392(VOUTP_FDSOV2Cmd_flg) -> bus_creator/392
  outpmodule/270(VOUTP_AmbColorSta4_enum) -> bus_creator/270
  bus_selector15/22 -> outpmodule/606(VVMC_ISOJerkLimit_mps3)  "<VVMC_ISOJerkLimit_mps3>"
  bus_selector2/135 -> outpmodule/138(VAPM_AVMparkingcancelTimeOut_flg)  "<VAPM_AVMparkingcancelTimeOut_flg>"
  outpmodule/421(VOUTP_sigClntTHvBattOut_C) -> bus_creator/421
  outpmodule/483(VOUTP_S1ID_raw32) -> bus_creator/483
  outpmodule/277(VOUTP_AmbBrightnessSta5_enum) -> bus_creator/277
  outpmodule/266(VOUTP_AmbODAENFlash_enum) -> bus_creator/266
  bus_selector2/64 -> outpmodule/67(VAPM_LRWhlRotDir_enum)  "<VAPM_LRWhlRotDir_enum>"
  outpmodule/608(VOUTP_DISCReqAcc_mps2) -> bus_creator/608
  outpmodule/427(VOUTP_ACSubMode_enum) -> bus_creator/427
  outpmodule/267(VOUTP_AmbColorSta1_enum) -> bus_creator/267
  outpmodule/265(VOUTP_AmbPwrWarnENFlash_enum) -> bus_creator/265
  outpmodule/263(VOUTP_AmbDimENFlash_enum) -> bus_creator/263
  bus_selector15/88 -> outpmodule/672(VVMC_CCCtrlSta_enum)  "<VVMC_CCCtrlSta_enum>"
  outpmodule/535(VOUTP_TqSourceRr_enum) -> bus_creator/535
  outpmodule/261(VOUTP_AmbFunENFlash_enum) -> bus_creator/261
  bus_selector3/39 -> outpmodule/204(VBCM_RoomLampH_flg)  "<VBCM_RoomLampH_flg>"
  outpmodule/260(VOUTP_UserNow_enum) -> bus_creator/260
  outpmodule/429(VOUTP_ACModeMem_enum) -> bus_creator/429
  outpmodule/259(VOUTP_fUnlockSingle_flg) -> bus_creator/259
  bus_selector3/94 -> outpmodule/259(VBCM_fUnlockSingle_flg)  "<VBCM_fUnlockSingle_flg>"
  outpmodule/257(VOUTP_LockAlarm_enum) -> bus_creator/257
  bus_selector2/144 -> outpmodule/147(VAPM_CAASSw_enum)  "<VAPM_CAASSw_enum>"
  outpmodule/255(VOUTP_AmbColorSta_enum) -> bus_creator/255
  outpmodule/467(VOUTP_RRPressIndi_enum) -> bus_creator/467
  outpmodule/256(VOUTP_AmbBrightSta_enum) -> bus_creator/256
  outpmodule/276(VOUTP_AmbBrightnessSta4_enum) -> bus_creator/276
  bus_selector3/64 -> outpmodule/229(VBCM_AmbLightColor5_enum)  "<VBCM_AmbLightColor5_enum>"
  bus_selector2/37 -> outpmodule/40(VAPM_USSStaFCL_flg)  "<VAPM_USSStaFCL_flg>"
  outpmodule/252(VOUTP_AmbLinkDriSta_flg) -> bus_creator/252
  bus_selector2/147 -> outpmodule/150(VAPM_IVIScreenTimeOut_flg)  "<VAPM_IVIScreenTimeOut_flg>"
  outpmodule/250(VOUTP_AmbWelEN_flg) -> bus_creator/250
  bus_selector15/83 -> outpmodule/667(VVMC_FCMLDWRequest_enum)  "<VVMC_FCMLDWRequest_enum>"
  outpmodule/246(VOUTP_LRLDCtrlCmd_pct) -> bus_creator/246
  outpmodule/588(VOUTP_MeterIndSpeed_raw32) -> bus_creator/588
  outpmodule/245(VOUTP_LPasCtrlCmd_pct) -> bus_creator/245
  bus_selector7/9 -> outpmodule/302(VNMM_WakeUp_enum)  "<VNMM_WakeUp_enum>"
  outpmodule/244(VOUTP_LDrvCtrlCmd_pct) -> bus_creator/244
  outpmodule/243(VOUTP_PTGInnerSW2_enum) -> bus_creator/243
  bus_selector2/138 -> outpmodule/141(VAPM_AVMParkingmode_enum)  "<VAPM_AVMParkingmode_enum>"
  outpmodule/241(VOUTP_RoomLampMode_flg) -> bus_creator/241
  outpmodule/489(VOUTP_S3L_enum) -> bus_creator/489
  outpmodule/240(VOUTP_MFRDNBrightReq_pct) -> bus_creator/240
  outpmodule/330(VOUTP_LVSysErrPwrOutErr_flg) -> bus_creator/330
  outpmodule/237(VOUTP_MFSWTri_flg) -> bus_creator/237
  outpmodule/239(VOUTP_FuelDoorPos_flg) -> bus_creator/239
  outpmodule/238(VOUTP_MirrorFlodPos_flg) -> bus_creator/238
  bus_selector2/1 -> outpmodule/4(VAPM_VehSpeed_kph)  "<VAPM_VehSpeed_kph>"
  outpmodule/275(VOUTP_AmbBrightnessSta3_enum) -> bus_creator/275
  outpmodule/235(VOUTP_IVIRST_flg) -> bus_creator/235
  outpmodule/232(VOUTP_SPTGDet_flg) -> bus_creator/232
  outpmodule/229(VOUTP_AmbLightColor5_enum) -> bus_creator/229
  outpmodule/225(VOUTP_AmbLightColor1_enum) -> bus_creator/225
  outpmodule/226(VOUTP_AmbLightColor2_enum) -> bus_creator/226
  outpmodule/223(VOUTP_AmbLightBrightness5_enum) -> bus_creator/223
  outpmodule/224(VOUTP_AmbLightBrightness6_enum) -> bus_creator/224
  outpmodule/222(VOUTP_AmbLightBrightness4_enum) -> bus_creator/222
  bus_selector2/58 -> outpmodule/61(VAPM_RRRawWhlSpeedV_flg)  "<VAPM_RRRawWhlSpeedV_flg>"
  bus_selector3/23 -> outpmodule/188(VBCM_LBeam_flg)  "<VBCM_LBeam_flg>"
  outpmodule/219(VOUTP_AmbLightBrightness1_enum) -> bus_creator/219
  outpmodule/215(VOUTP_AmbLightBreath3_enum) -> bus_creator/215
  outpmodule/214(VOUTP_AmbLightBreath2_enum) -> bus_creator/214
  bus_selector15/87 -> outpmodule/671(VVMC_TimeGapCalcu_s)  "<VVMC_TimeGapCalcu_s>"
  outpmodule/211(VOUTP_WasherCtrl_enum) -> bus_creator/211
  outpmodule/210(VOUTP_RrWiper_flg) -> bus_creator/210
  outpmodule/327(VOUTP_PwrDownReq_enum) -> bus_creator/327
  outpmodule/208(VOUTP_FrWiperL_flg) -> bus_creator/208
  bus_selector15/93 -> outpmodule/677(VVMC_APSDecReq_mps2)  "<VVMC_APSDecReq_mps2>"
  outpmodule/205(VOUTP_RoomLampL_flg) -> bus_creator/205
  bus_selector15/71 -> outpmodule/655(VVMC_LVDADisabled_flg)  "<VVMC_LVDADisabled_flg>"
  outpmodule/200(VOUTP_BCMBuzzerReq_flg) -> bus_creator/200
  outpmodule/199(VOUTP_RTurnLP_flg) -> bus_creator/199
  bus_selector15/23 -> outpmodule/607(VVMC_ACCRequiredAccel_mps2)  "<VVMC_ACCRequiredAccel_mps2>"
  outpmodule/274(VOUTP_AmbBrightnessSta2_enum) -> bus_creator/274
  outpmodule/191(VOUTP_BrakeLamp_flg) -> bus_creator/191
  outpmodule/188(VOUTP_LBeam_flg) -> bus_creator/188
  outpmodule/189(VOUTP_HBeam_flg) -> bus_creator/189
  bus_selector11/44 -> outpmodule/485(VTPM_S3ID_raw32)  "<VTPM_S3ID_raw32>"
  outpmodule/517(VOUTP_WriteChkLRID_raw) -> bus_creator/517
  outpmodule/262(VOUTP_AmbWelENFlash_enum) -> bus_creator/262
  bus_selector3/92 -> outpmodule/257(VBCM_LockAlarm_enum)  "<VBCM_LockAlarm_enum>"
  outpmodule/184(VOUTP_CTDLockSW_flg) -> bus_creator/184
  outpmodule/186(VOUTP_DimmerEN_flg) -> bus_creator/186
  outpmodule/183(VOUTP_DoorLockIND_flg) -> bus_creator/183
  outpmodule/180(VOUTP_RrChargingDoorCtrl_enum) -> bus_creator/180
  bus_selector15/30 -> outpmodule/614(VVMC_LKATOIAct_enum)  "<VVMC_LKATOIAct_enum>"
  outpmodule/176(VOUTP_RLDoorSW_flg) -> bus_creator/176
  bus_selector15/21 -> outpmodule/605(VVMC_ISODecLimit_mps2)  "<VVMC_ISODecLimit_mps2>"
  outpmodule/174(VOUTP_DrDoorSW_flg) -> bus_creator/174
  bus_selector15/39 -> outpmodule/623(VVMC_TimeGapLevel_enum)  "<VVMC_TimeGapLevel_enum>"
  outpmodule/171(VOUTP_AntitheftSeatFlod_flg) -> bus_creator/171
  outpmodule/172(VOUTP_HoodSW_flg) -> bus_creator/172
  bus_selector15/27 -> outpmodule/611(VVMC_ADASLKASta_enum)  "<VVMC_ADASLKASta_enum>"
  outpmodule/169(VOUTP_AllDoorSW_flg) -> bus_creator/169
  outpmodule/242(VOUTP_IVIPTGUSStaSW_flg) -> bus_creator/242
  bus_selector11/25 -> outpmodule/466(VTPM_LRPressIndi_enum)  "<VTPM_LRPressIndi_enum>"
  outpmodule/168(VOUTP_HornCtrl_flg) -> bus_creator/168
  outpmodule/227(VOUTP_AmbLightColor3_enum) -> bus_creator/227
  bus_selector3/13 -> outpmodule/178(VBCM_LockSetting_flg)  "<VBCM_LockSetting_flg>"
  outpmodule/230(VOUTP_AmbLightColor6_enum) -> bus_creator/230
  outpmodule/554(VOUTP_FrEDUAvailBrkRgnTqV_flg) -> bus_creator/554
  outpmodule/166(VOUTP_AntitheftSta_enum) -> bus_creator/166
  outpmodule/161(VOUTP_APSExitCondition_enum) -> bus_creator/161
  outpmodule/196(VOUTP_RBSD_flg) -> bus_creator/196
  bus_selector15/24 -> outpmodule/608(VVMC_DISCReqAcc_mps2)  "<VVMC_DISCReqAcc_mps2>"
  outpmodule/158(VOUTP_APSRQDisplay_enum) -> bus_creator/158
  outpmodule/157(VOUTP_APSProgressPCT_pct) -> bus_creator/157
  outpmodule/538(VOUTP_EVDriveMode_enum) -> bus_creator/538
  outpmodule/154(VOUTP_TCSActiveTimeOut_flg) -> bus_creator/154
  outpmodule/578(VOUTP_SpdCtrlMode_enum) -> bus_creator/578
  bus_selector4/2 -> outpmodule/286(VDHP_EAPS1MIN_pct)  "<VDHP_EAPS1MIN_pct>"
  outpmodule/152(VOUTP_ABSActiveTimeOut_flg) -> bus_creator/152
  bus_selector15/26 -> outpmodule/610(VVMC_LateralCtrl_flg)  "<VVMC_LateralCtrl_flg>"
  outpmodule/151(VOUTP_ABSActive_flg) -> bus_creator/151
  outpmodule/436(VOUTP_ACForceOFF_flg) -> bus_creator/436
  outpmodule/149(VOUTP_IVIScreen_enum) -> bus_creator/149
  outpmodule/145(VOUTP_IVIStatus_flg) -> bus_creator/145
  bus_selector3/85 -> outpmodule/250(VBCM_AmbWelEN_flg)  "<VBCM_AmbWelEN_flg>"
  outpmodule/143(VOUTP_AVMErrSTA_flg) -> bus_creator/143
  outpmodule/138(VOUTP_AVMparkingcancelTimeOut_flg) -> bus_creator/138
  outpmodule/139(VOUTP_AVMparkingexcute_enum) -> bus_creator/139
  bus_selector12/46 -> outpmodule/578(VTQD_SpdCtrlMode_enum)  "<VTQD_SpdCtrlMode_enum>"
  outpmodule/136(VOUTP_EPBStaTimeOut_flg) -> bus_creator/136
  outpmodule/490(VOUTP_S4L_enum) -> bus_creator/490
  outpmodule/130(VOUTP_EPBExtReleaseAvailTimeOut_flg) -> bus_creator/130
  outpmodule/128(VOUTP_ESCAPSStaTimeOut_flg) -> bus_creator/128
  bus_selector3/2 -> outpmodule/167(VBCM_TailgateRemote_enum)  "<VBCM_TailgateRemote_enum>"
  outpmodule/129(VOUTP_EPBExtReleaseAvail_flg) -> bus_creator/129
  outpmodule/127(VOUTP_ESCAPSSta_enum) -> bus_creator/127
  bus_selector3/42 -> outpmodule/207(VBCM_TailgateHDSW_flg)  "<VBCM_TailgateHDSW_flg>"
  outpmodule/126(VOUTP_ESCStandstillTimeOut_flg) -> bus_creator/126
  outpmodule/249(VOUTP_AmbFunEN_flg) -> bus_creator/249
  bus_selector7/2 -> outpmodule/295(VNMM_NMmTxReq_flg)  "<VNMM_NMmTxReq_flg>"
  outpmodule/121(VOUTP_BrkSwSta_flg) -> bus_creator/121
  outpmodule/193(VOUTP_LDRL_flg) -> bus_creator/193
  bus_selector15/40 -> outpmodule/624(VVMC_ACCJerkUpperLimit_mps3)  "<VVMC_ACCJerkUpperLimit_mps3>"
  outpmodule/35(VOUTP_USSStaFMR_flg) -> bus_creator/35
  bus_selector15/68 -> outpmodule/652(VVMC_ADASLDWMute_flg)  "<VVMC_ADASLDWMute_flg>"
  outpmodule/27(VOUTP_PASAFML_enum) -> bus_creator/27
  outpmodule/23(VOUTP_PASARML_enum) -> bus_creator/23
  outpmodule/455(VOUTP_RFSensorFail_flg) -> bus_creator/455
  outpmodule/20(VOUTP_APSDFLL_cm) -> bus_creator/20
  outpmodule/334(VOUTP_LVChrgHoldTtimer_s) -> bus_creator/334
  outpmodule/21(VOUTP_PASAFCL_enum) -> bus_creator/21
  bus_selector3/31 -> outpmodule/196(VBCM_RBSD_flg)  "<VBCM_RBSD_flg>"
  outpmodule/415(VOUTP_CCUSyncLampSts_flg) -> bus_creator/415
  outpmodule/18(VOUTP_APSDRLL_cm) -> bus_creator/18
  bus_selector3/44 -> outpmodule/209(VBCM_FrWiperH_flg)  "<VBCM_FrWiperH_flg>"
  outpmodule/19(VOUTP_APSDFLR_cm) -> bus_creator/19
  outpmodule/523(VOUTP_Flashchkdatavalid_enum) -> bus_creator/523
  outpmodule/17(VOUTP_APSDRLR_cm) -> bus_creator/17
  bus_selector8/10 -> outpmodule/315(VPMM_PowerSta_enum)  "<VPMM_PowerSta_enum>"
  outpmodule/198(VOUTP_LTurnLP_flg) -> bus_creator/198
  outpmodule/16(VOUTP_PASDFCL_cm) -> bus_creator/16
  outpmodule/14(VOUTP_PASDFML_cm) -> bus_creator/14
  outpmodule/325(VOUTP_TCountSta_enum) -> bus_creator/325
  outpmodule/155(VOUTP_DriverSeatBeltCmd_flg) -> bus_creator/155
  outpmodule/12(VOUTP_PASDRCL_cm) -> bus_creator/12
  bus_selector9/35 -> outpmodule/388(VSYS_AcoreRebootCmdACK_flg)  "<VSYS_AcoreRebootCmdACK_flg>"
  outpmodule/9(VOUTP_PASDRMR_cm) -> bus_creator/9
  outpmodule/24(VOUTP_PASARCR_enum) -> bus_creator/24
  outpmodule/529(VOUTP_FlashS2ID_raw) -> bus_creator/529
  outpmodule/332(VOUTP_PwrStaONTOPopReq_flg) -> bus_creator/332
  outpmodule/216(VOUTP_AmbLightBreath4_enum) -> bus_creator/216
  outpmodule/7(VOUTP_FSOffSwTimeOut_flg) -> bus_creator/7
  bus_selector8/9 -> outpmodule/314(VPMM_HVSysReadyToCharge_enum)  "<VPMM_HVSysReadyToCharge_enum>"
  bus_selector2/118 -> outpmodule/121(VAPM_BrkSwSta_flg)  "<VAPM_BrkSwSta_flg>"
  outpmodule/5(VOUTP_VehSpeedTimeOut_flg) -> bus_creator/5
  outpmodule/3(VOUTP_VehHVPwrAvail4THCM_W) -> bus_creator/3
  outpmodule/4(VOUTP_VehSpeed_kph) -> bus_creator/4
  outpmodule/1(VOUTP_HVTHCMSysAvail_enum) -> bus_creator/1
  bus_selector3/46 -> outpmodule/211(VBCM_WasherCtrl_enum)  "<VBCM_WasherCtrl_enum>"
  outpmodule/499(VOUTP_S2WheelDebugALTU_pct) -> bus_creator/499
  outpmodule/36(VOUTP_USSStaFML_flg) -> bus_creator/36
  outpmodule/37(VOUTP_USSStaFLR_flg) -> bus_creator/37
  bus_selector2/13 -> outpmodule/16(VAPM_PASDFCL_cm)  "<VAPM_PASDFCL_cm>"
  outpmodule/443(VOUTP_RFBatWarn_flg) -> bus_creator/443
  outpmodule/190(VOUTP_RrFogLamp_flg) -> bus_creator/190
  outpmodule/170(VOUTP_BCMDoorLockSta_flg) -> bus_creator/170
  outpmodule/110(VOUTP_LongAccelTimeOut_flg) -> bus_creator/110
  outpmodule/108(VOUTP_LatAccelTimeOut_flg) -> bus_creator/108
  outpmodule/185(VOUTP_Dimmer_pct) -> bus_creator/185
  outpmodule/114(VOUTP_YawRateVTimeOut_flg) -> bus_creator/114
  outpmodule/113(VOUTP_YawRateV_flg) -> bus_creator/113
  bus_selector11/38 -> outpmodule/479(VTPM_LFSensorMode_flg)  "<VTPM_LFSensorMode_flg>"
  outpmodule/105(VOUTP_YawRate_degps) -> bus_creator/105
  bus_selector12/41 -> outpmodule/573(VTQD_ActParkRequest_flg)  "<VTQD_ActParkRequest_flg>"
  outpmodule/106(VOUTP_YawRateTimeOut_flg) -> bus_creator/106
  outpmodule/104(VOUTP_GRADETimeOut_flg) -> bus_creator/104
  outpmodule/617(VOUTP_AEBVehHoldReq_flg) -> bus_creator/617
  bus_selector11/28 -> outpmodule/469(VTPM_LFWheelTmpIndi_flg)  "<VTPM_LFWheelTmpIndi_flg>"
  outpmodule/179(VOUTP_FrChargingDoorCtrl_enum) -> bus_creator/179
  outpmodule/103(VOUTP_GRADE_Deg) -> bus_creator/103
  outpmodule/150(VOUTP_IVIScreenTimeOut_flg) -> bus_creator/150
  outpmodule/555(VOUTP_RrEDUSpdValid_flg) -> bus_creator/555
  outpmodule/100(VOUTP_SASCALTimeOut_flg) -> bus_creator/100
  outpmodule/470(VOUTP_RFWheelTmpIndi_flg) -> bus_creator/470
  outpmodule/614(VOUTP_LKATOIAct_enum) -> bus_creator/614
  outpmodule/99(VOUTP_SASCAL_flg) -> bus_creator/99
  outpmodule/98(VOUTP_SASSpeedValidTimeOut_flg) -> bus_creator/98
  outpmodule/528(VOUTP_FlashS1ID_raw) -> bus_creator/528
  outpmodule/374(VOUTP_Dash2_cnt) -> bus_creator/374
  outpmodule/159(VOUTP_APSSWVer_enum) -> bus_creator/159
  outpmodule/371(VOUTP_Dash1_cnt) -> bus_creator/371
  outpmodule/370(VOUTP_Variation_cnt) -> bus_creator/370
  outpmodule/328(VOUTP_LowSOCWarn_enum) -> bus_creator/328
  outpmodule/10(VOUTP_PASDRML_cm) -> bus_creator/10
  outpmodule/369(VOUTP_Country2_cnt) -> bus_creator/369
  outpmodule/594(VOUTP_FeatReqSpd_kph) -> bus_creator/594
  outpmodule/543(VOUTP_FrRgnDecrSta_flg) -> bus_creator/543
  outpmodule/366(VOUTP_Patch1_cnt) -> bus_creator/366
  outpmodule/273(VOUTP_AmbBrightnessSta1_enum) -> bus_creator/273
  outpmodule/365(VOUTP_Minor2_cnt) -> bus_creator/365
  outpmodule/363(VOUTP_Major2_cnt) -> bus_creator/363
  bus_selector2/109 -> outpmodule/112(VAPM_MCPressureTimeOut_flg)  "<VAPM_MCPressureTimeOut_flg>"
  outpmodule/361(VOUTP_ECU2_cnt) -> bus_creator/361
  outpmodule/426(VOUTP_sigCbnAirT_C) -> bus_creator/426
  outpmodule/359(VOUTP_CarModel3_cnt) -> bus_creator/359
  bus_selector2/50 -> outpmodule/53(VAPM_RRRawWhlSpeed_kph)  "<VAPM_RRRawWhlSpeed_kph>"
  outpmodule/461(VOUTP_RRWheelDebug_flg) -> bus_creator/461
  outpmodule/357(VOUTP_CarModel1_cnt) -> bus_creator/357
  bus_selector2/140 -> outpmodule/143(VAPM_AVMErrSTA_flg)  "<VAPM_AVMErrSTA_flg>"
  outpmodule/353(VOUTP_OTAPwrReqStdChkSta_enum) -> bus_creator/353
  bus_selector15/84 -> outpmodule/668(VVMC_FCMLDWFault_flg)  "<VVMC_FCMLDWFault_flg>"
  outpmodule/352(VOUTP_OTAPwrReqOFFChkSta_enum) -> bus_creator/352
  outpmodule/348(VOUTP_CtrlDrPwrStbA2_flg) -> bus_creator/348
  bus_selector2/152 -> outpmodule/155(VAPM_DriverSeatBeltCmd_flg)  "<VAPM_DriverSeatBeltCmd_flg>"
  outpmodule/438(VOUTP_AirIntenZone1M_enum) -> bus_creator/438
  outpmodule/559(VOUTP_FrRgnPermSta_flg) -> bus_creator/559
  outpmodule/134(VOUTP_EPBErrStaTimeOut_flg) -> bus_creator/134
  bus_selector8/13 -> outpmodule/318(VPMM_SysPowerMode_enum)  "<VPMM_SysPowerMode_enum>"
  outpmodule/460(VOUTP_RFWheelDebug_flg) -> bus_creator/460
  outpmodule/350(VOUTP_Sched_ChgTOSta_enum) -> bus_creator/350
  outpmodule/346(VOUTP_CtrlFrEDUINVERTER_flg) -> bus_creator/346
  outpmodule/264(VOUTP_AmbLinkDriStaFlash_enum) -> bus_creator/264
  outpmodule/345(VOUTP_CtrlFrBMSCCUCIR_flg) -> bus_creator/345
  bus_selector8/2 -> outpmodule/307(VPMM_PowerDownState_enum)  "<VPMM_PowerDownState_enum>"
  outpmodule/323(VOUTP_PwrStaSelect_enum) -> bus_creator/323
  bus_selector10/36 -> outpmodule/425(VTHC_sigAmbAirT_C)  "<VTHC_sigAmbAirT_C>"
  outpmodule/526(VOUTP_unlearnSfailvalid_enum) -> bus_creator/526
  outpmodule/581(VOUTP_FrTMTqReq_Nm) -> bus_creator/581
  outpmodule/195(VOUTP_LBSD_flg) -> bus_creator/195
  outpmodule/342(VOUTP_LVSilentChrgLv_enum) -> bus_creator/342
  outpmodule/131(VOUTP_EPBExtApplyAvail_flg) -> bus_creator/131
  outpmodule/560(VOUTP_RrRgnPermSta_flg) -> bus_creator/560
  outpmodule/343(VOUTP_CtrlFrPwrStbA1P_flg) -> bus_creator/343
  bus_selector2/41 -> outpmodule/44(VAPM_ModOperation_enum)  "<VAPM_ModOperation_enum>"
  outpmodule/379(VOUTP_SHA5_cnt) -> bus_creator/379
  bus_selector2/143 -> outpmodule/146(VAPM_IVIStatusTimeOut_flg)  "<VAPM_IVIStatusTimeOut_flg>"
  outpmodule/398(VOUTP_FDTWVCmd_pct) -> bus_creator/398
  outpmodule/377(VOUTP_SHA3_cnt) -> bus_creator/377
  bus_selector15/81 -> outpmodule/665(VVMC_ADASLanecurveR_raw32)  "<VVMC_ADASLanecurveR_raw32>"
  outpmodule/85(VOUTP_RRPulseCount_enum) -> bus_creator/85
  outpmodule/218(VOUTP_AmbLightBreath6_enum) -> bus_creator/218
  outpmodule/77(VOUTP_RRPulseCountV_flg) -> bus_creator/77
  bus_selector3/6 -> outpmodule/171(VBCM_AntitheftSeatFlod_flg)  "<VBCM_AntitheftSeatFlod_flg>"
  outpmodule/616(VOUTP_ADASFaultSta_flg) -> bus_creator/616
  outpmodule/144(VOUTP_AVMErrSTATimeOut_flg) -> bus_creator/144
  outpmodule/75(VOUTP_LRPulseCountV_flg) -> bus_creator/75
  bus_selector15/4 -> outpmodule/588(VVMC_MeterIndSpeed_raw32)  "<VVMC_MeterIndSpeed_raw32>"
  bus_selector2/121 -> outpmodule/124(VAPM_BrkSwVTimeOut_flg)  "<VAPM_BrkSwVTimeOut_flg>"
  outpmodule/514(VOUTP_RRPindi_enum) -> bus_creator/514
  outpmodule/194(VOUTP_RDRL_flg) -> bus_creator/194
  outpmodule/38(VOUTP_USSStaFLL_flg) -> bus_creator/38
  outpmodule/403(VOUTP_FDEWP2Cmd_enum) -> bus_creator/403
  outpmodule/228(VOUTP_AmbLightColor4_enum) -> bus_creator/228
  outpmodule/358(VOUTP_CarModel2_cnt) -> bus_creator/358
  outpmodule/73(VOUTP_RFPulseCountV_flg) -> bus_creator/73
  outpmodule/72(VOUTP_LFPulseCountVTimeOut_flg) -> bus_creator/72
  outpmodule/71(VOUTP_LFPulseCountV_flg) -> bus_creator/71
  outpmodule/70(VOUTP_RRWhlRotDirTimeOut_flg) -> bus_creator/70
  outpmodule/69(VOUTP_RRWhlRotDir_enum) -> bus_creator/69
  outpmodule/530(VOUTP_FlashS3ID_raw) -> bus_creator/530
  outpmodule/380(VOUTP_SHA6_cnt) -> bus_creator/380
  outpmodule/68(VOUTP_LRWhlRotDirTimeOut_flg) -> bus_creator/68
  outpmodule/67(VOUTP_LRWhlRotDir_enum) -> bus_creator/67
  outpmodule/66(VOUTP_RFWhlRotDirTimeOut_flg) -> bus_creator/66
  outpmodule/351(VOUTP_PwrReq_OTA_enum) -> bus_creator/351
  outpmodule/63(VOUTP_LFWhlRotDir_enum) -> bus_creator/63
  outpmodule/234(VOUTP_FollowMe_flg) -> bus_creator/234
  bus_selector11/34 -> outpmodule/475(VTPM_RFWheelPSW_raw8)  "<VTPM_RFWheelPSW_raw8>"
  bus_selector2/120 -> outpmodule/123(VAPM_BrkSwV_flg)  "<VAPM_BrkSwV_flg>"
  outpmodule/112(VOUTP_MCPressureTimeOut_flg) -> bus_creator/112
  outpmodule/61(VOUTP_RRRawWhlSpeedV_flg) -> bus_creator/61
  outpmodule/453(VOUTP_RRWheelTemp_C) -> bus_creator/453
  outpmodule/160(VOUTP_APSHWVer_enum) -> bus_creator/160
  bus_selector8/1 -> outpmodule/306(VPMM_PowerUpState_enum)  "<VPMM_PowerUpState_enum>"
  bus_selector6/2 -> outpmodule/291(VDSC_DISCTargetSpd_kph)  "<VDSC_DISCTargetSpd_kph>"
  outpmodule/60(VOUTP_LRRawWhlSpeedVTimeOut_flg) -> bus_creator/60
  bus_selector3/47 -> outpmodule/212(VBCM_WiperFixMode_flg)  "<VBCM_WiperFixMode_flg>"
  bus_selector3/105 -> outpmodule/270(VBCM_AmbColorSta4_enum)  "<VBCM_AmbColorSta4_enum>"
  outpmodule/59(VOUTP_LRRawWhlSpeedV_flg) -> bus_creator/59
  outpmodule/55(VOUTP_LFRawWhlSpeedV_flg) -> bus_creator/55
  outpmodule/53(VOUTP_RRRawWhlSpeed_kph) -> bus_creator/53
  outpmodule/444(VOUTP_LRBatWarn_flg) -> bus_creator/444
  outpmodule/181(VOUTP_CrashDetd_flg) -> bus_creator/181
  outpmodule/201(VOUTP_MirrorCtrl_enum) -> bus_creator/201
  outpmodule/52(VOUTP_LRRawWhlSpeedTimeOut_flg) -> bus_creator/52
  outpmodule/6(VOUTP_FSOffSw_enum) -> bus_creator/6
  outpmodule/50(VOUTP_RFRawWhlSpeedTimeOut_flg) -> bus_creator/50
  bus_selector3/60 -> outpmodule/225(VBCM_AmbLightColor1_enum)  "<VBCM_AmbLightColor1_enum>"
  bus_selector2/45 -> outpmodule/48(VAPM_LFRawWhlSpeedTimeOut_flg)  "<VAPM_LFRawWhlSpeedTimeOut_flg>"
  outpmodule/48(VOUTP_LFRawWhlSpeedTimeOut_flg) -> bus_creator/48
  bus_selector15/70 -> outpmodule/654(VVMC_ADASLFCHandsOffWarning_enum)  "<VVMC_ADASLFCHandsOffWarning_enum>"
  outpmodule/49(VOUTP_RFRawWhlSpeed_kph) -> bus_creator/49
  bus_selector3/8 -> outpmodule/173(VBCM_TailgateSW_flg)  "<VBCM_TailgateSW_flg>"
  outpmodule/47(VOUTP_LFRawWhlSpeed_kph) -> bus_creator/47
  bus_selector2/61 -> outpmodule/64(VAPM_LFWhlRotDirTimeOut_flg)  "<VAPM_LFWhlRotDirTimeOut_flg>"
  bus_selector11/23 -> outpmodule/464(VTPM_LFPressIndi_enum)  "<VTPM_LFPressIndi_enum>"
  outpmodule/44(VOUTP_ModOperation_enum) -> bus_creator/44
  outpmodule/43(VOUTP_StaFSya_flg) -> bus_creator/43
  bus_selector3/86 -> outpmodule/251(VBCM_AmbDimEN_flg)  "<VBCM_AmbDimEN_flg>"
  outpmodule/433(VOUTP_FaceM_flg) -> bus_creator/433
  outpmodule/212(VOUTP_WiperFixMode_flg) -> bus_creator/212
  outpmodule/42(VOUTP_SNSRLayout_enum) -> bus_creator/42
  bus_selector2/128 -> outpmodule/131(VAPM_EPBExtApplyAvail_flg)  "<VAPM_EPBExtApplyAvail_flg>"
  outpmodule/40(VOUTP_USSStaFCL_flg) -> bus_creator/40
  outpmodule/41(VOUTP_Chime_enum) -> bus_creator/41
  outpmodule/388(VOUTP_AcoreRebootCmdACK_flg) -> bus_creator/388
  bus_selector2/93 -> outpmodule/96(VAPM_SASSpeedTimeOut_flg)  "<VAPM_SASSpeedTimeOut_flg>"
  bus_selector2/91 -> outpmodule/94(VAPM_SASAngleTimeOut_flg)  "<VAPM_SASAngleTimeOut_flg>"
  outpmodule/111(VOUTP_MCPressure_bar) -> bus_creator/111
  bus_selector2/92 -> outpmodule/95(VAPM_SASSpeed_degps)  "<VAPM_SASSpeed_degps>"
  bus_selector2/88 -> outpmodule/91(VAPM_EPSAOIControl_enum)  "<VAPM_EPSAOIControl_enum>"
  bus_selector2/142 -> outpmodule/145(VAPM_IVIStatus_flg)  "<VAPM_IVIStatus_flg>"
  bus_selector2/87 -> outpmodule/90(VAPM_DriIntendTimeOut_flg)  "<VAPM_DriIntendTimeOut_flg>"
  outpmodule/280(VOUTP_DimSwSta_flg) -> bus_creator/280
  outpmodule/463(VOUTP_TPMSCaliButtAllow_flg) -> bus_creator/463
  outpmodule/347(VOUTP_HWResetSta_enum) -> bus_creator/347
  outpmodule/597(VOUTP_FrontRearSlipRatioCtrl_flg) -> bus_creator/597
  outpmodule/115(VOUTP_LatAccelV_flg) -> bus_creator/115
  outpmodule/78(VOUTP_RRPulseCountVTimeOut_flg) -> bus_creator/78
  bus_selector2/85 -> outpmodule/88(VAPM_ShifterHandleCmdTimeOut_flg)  "<VAPM_ShifterHandleCmdTimeOut_flg>"
  outpmodule/133(VOUTP_EPBErrSta_enum) -> bus_creator/133
  bus_selector2/82 -> outpmodule/85(VAPM_RRPulseCount_enum)  "<VAPM_RRPulseCount_enum>"
  bus_selector2/84 -> outpmodule/87(VAPM_ShifterHandleCmd_enum)  "<VAPM_ShifterHandleCmd_enum>"
  bus_selector10/7 -> outpmodule/396(VTHC_FDSOTXVCmd_flg)  "<VTHC_FDSOTXVCmd_flg>"
  outpmodule/310(VOUTP_ActiveDischargeReq_flg) -> bus_creator/310
  bus_selector2/83 -> outpmodule/86(VAPM_RRPulseCountTimeOut_flg)  "<VAPM_RRPulseCountTimeOut_flg>"
  outpmodule/165(VOUTP_CAASSta_enum) -> bus_creator/165
  bus_selector2/80 -> outpmodule/83(VAPM_LRPulseCount_enum)  "<VAPM_LRPulseCount_enum>"
  outpmodule/107(VOUTP_LatAccel_Gps) -> bus_creator/107
  outpmodule/502(VOUTP_ID1messageALTU_raw8) -> bus_creator/502
  bus_selector2/76 -> outpmodule/79(VAPM_LFPulseCount_enum)  "<VAPM_LFPulseCount_enum>"
  outpmodule/25(VOUTP_PASARCL_enum) -> bus_creator/25
  bus_selector2/77 -> outpmodule/80(VAPM_LFPulseCountTimeOut_flg)  "<VAPM_LFPulseCountTimeOut_flg>"
  outpmodule/56(VOUTP_LFRawWhlSpeedVTimeOut_flg) -> bus_creator/56
  bus_selector2/75 -> outpmodule/78(VAPM_RRPulseCountVTimeOut_flg)  "<VAPM_RRPulseCountVTimeOut_flg>"
  outpmodule/32(VOUTP_USSStaRLL_flg) -> bus_creator/32
  bus_selector7/5 -> outpmodule/298(VNMM_ErrorState_enum)  "<VNMM_ErrorState_enum>"
  outpmodule/400(VOUTP_CoolgFanActDuty_pct) -> bus_creator/400
  bus_selector15/72 -> outpmodule/656(VVMC_LVDAMuteSta_enum)  "<VVMC_LVDAMuteSta_enum>"
  outpmodule/80(VOUTP_LFPulseCountTimeOut_flg) -> bus_creator/80
  bus_selector2/74 -> outpmodule/77(VAPM_RRPulseCountV_flg)  "<VAPM_RRPulseCountV_flg>"
  outpmodule/203(VOUTP_RrDefog_flg) -> bus_creator/203
  bus_selector2/103 -> outpmodule/106(VAPM_YawRateTimeOut_flg)  "<VAPM_YawRateTimeOut_flg>"
  outpmodule/54(VOUTP_RRRawWhlSpeedTimeOut_flg) -> bus_creator/54
  bus_selector2/102 -> outpmodule/105(VAPM_YawRate_degps)  "<VAPM_YawRate_degps>"
  outpmodule/326(VOUTP_PwrUpReq_enum) -> bus_creator/326
  bus_selector2/100 -> outpmodule/103(VAPM_GRADE_Deg)  "<VAPM_GRADE_Deg>"
  outpmodule/354(VOUTP_HWVer1_cnt) -> bus_creator/354
  outpmodule/561(VOUTP_FrIdcMin_A) -> bus_creator/561
  outpmodule/217(VOUTP_AmbLightBreath5_enum) -> bus_creator/217
  bus_selector2/101 -> outpmodule/104(VAPM_GRADETimeOut_flg)  "<VAPM_GRADETimeOut_flg>"
  outpmodule/33(VOUTP_USSStaRCR_flg) -> bus_creator/33
  BVMC_outputs/1 -> bus_selector15/1
  bus_selector2/94 -> outpmodule/97(VAPM_SASSpeedValid_flg)  "<VAPM_SASSpeedValid_flg>"
  outpmodule/248(VOUTP_APMDoorControlSta_flg) -> bus_creator/248
  bus_selector12/45 -> outpmodule/577(VTQD_FDCVCURegenMode_enum)  "<VTQD_FDCVCURegenMode_enum>"
  bus_selector2/98 -> outpmodule/101(VAPM_SASV_flg)  "<VAPM_SASV_flg>"
  outpmodule/355(VOUTP_HWVer2_cnt) -> bus_creator/355
  outpmodule/412(VOUTP_CCUACLampSts_flg) -> bus_creator/412
  outpmodule/251(VOUTP_AmbDimEN_flg) -> bus_creator/251
  outpmodule/29(VOUTP_USSStaRMR_flg) -> bus_creator/29
  bus_selector2/99 -> outpmodule/102(VAPM_SASVTimeOut_flg)  "<VAPM_SASVTimeOut_flg>"
  outpmodule/595(VOUTP_JerkPCT_pct) -> bus_creator/595
  outpmodule/269(VOUTP_AmbColorSta3_enum) -> bus_creator/269
  outpmodule/272(VOUTP_AmbColorSta7_enum) -> bus_creator/272
  bus_selector2/32 -> outpmodule/35(VAPM_USSStaFMR_flg)  "<VAPM_USSStaFMR_flg>"
  outpmodule/122(VOUTP_BrkSwStaTimeOut_flg) -> bus_creator/122
  bus_selector2/36 -> outpmodule/39(VAPM_USSStaFCR_flg)  "<VAPM_USSStaFCR_flg>"
  outpmodule/291(VOUTP_DISCTargetSpd_kph) -> bus_creator/291
  bus_selector2/68 -> outpmodule/71(VAPM_LFPulseCountV_flg)  "<VAPM_LFPulseCountV_flg>"
  outpmodule/550(VOUTP_RrEDURolRgnTq_Nm) -> bus_creator/550
  outpmodule/182(VOUTP_CTDCtrl_enum) -> bus_creator/182
  outpmodule/76(VOUTP_LRPulseCountVTimeOut_flg) -> bus_creator/76
  bus_selector9/13 -> outpmodule/366(VSYS_Patch1_cnt)  "<VSYS_Patch1_cnt>"
  bus_selector9/31 -> outpmodule/384(VSYS_FdcSlpReqRisingEdge_flg)  "<VSYS_FdcSlpReqRisingEdge_flg>"
  outpmodule/456(VOUTP_LRSensorFail_flg) -> bus_creator/456
  bus_selector9/12 -> outpmodule/365(VSYS_Minor2_cnt)  "<VSYS_Minor2_cnt>"
  bus_selector2/72 -> outpmodule/75(VAPM_LRPulseCountV_flg)  "<VAPM_LRPulseCountV_flg>"
  outpmodule/11(VOUTP_PASDRCR_cm) -> bus_creator/11
  bus_selector9/14 -> outpmodule/367(VSYS_Patch2_cnt)  "<VSYS_Patch2_cnt>"
  bus_selector9/9 -> outpmodule/362(VSYS_Major1_cnt)  "<VSYS_Major1_cnt>"
  bus_selector9/8 -> outpmodule/361(VSYS_ECU2_cnt)  "<VSYS_ECU2_cnt>"
  bus_selector15/54 -> outpmodule/638(VVMC_ACCObjDstLvl_enum)  "<VVMC_ACCObjDstLvl_enum>"
  bus_selector9/10 -> outpmodule/363(VSYS_Major2_cnt)  "<VSYS_Major2_cnt>"
  outpmodule/192(VOUTP_ReverseLamp_flg) -> bus_creator/192
  bus_selector15/16 -> outpmodule/600(VVMC_LatAccCtrl_flg)  "<VVMC_LatAccCtrl_flg>"
  bus_selector9/4 -> outpmodule/357(VSYS_CarModel1_cnt)  "<VSYS_CarModel1_cnt>"
  bus_selector9/3 -> outpmodule/356(VSYS_HWVer3_cnt)  "<VSYS_HWVer3_cnt>"
  outpmodule/590(VOUTP_VMCACCCtrlAvail_flg) -> bus_creator/590
  bus_selector9/2 -> outpmodule/355(VSYS_HWVer2_cnt)  "<VSYS_HWVer2_cnt>"
  bus_selector2/105 -> outpmodule/108(VAPM_LatAccelTimeOut_flg)  "<VAPM_LatAccelTimeOut_flg>"
  bus_selector15/7 -> outpmodule/591(VVMC_VMCCCCtrlAvail_flg)  "<VVMC_VMCCCCtrlAvail_flg>"
  outpmodule/146(VOUTP_IVIStatusTimeOut_flg) -> bus_creator/146
  bus_selector10/20 -> outpmodule/409(VTHC_BatteryMode_enum)  "<VTHC_BatteryMode_enum>"
  BPMM_outputs/1 -> bus_selector8/1
  bus_selector8/47 -> outpmodule/352(VPMM_OTAPwrReqOFFChkSta_enum)  "<VPMM_OTAPwrReqOFFChkSta_enum>"
  bus_selector8/48 -> outpmodule/353(VPMM_OTAPwrReqStdChkSta_enum)  "<VPMM_OTAPwrReqStdChkSta_enum>"
  bus_selector8/46 -> outpmodule/351(VPMM_PwrReq_OTA_enum)  "<VPMM_PwrReq_OTA_enum>"
  outpmodule/375(VOUTP_SHA1_cnt) -> bus_creator/375
  outpmodule/175(VOUTP_PsDoorSW_flg) -> bus_creator/175
  bus_selector8/45 -> outpmodule/350(VPMM_Sched_ChgTOSta_enum)  "<VPMM_Sched_ChgTOSta_enum>"
  bus_selector8/42 -> outpmodule/347(VPMM_HWResetSta_enum)  "<VPMM_HWResetSta_enum>"
  bus_selector11/20 -> outpmodule/461(VTPM_RRWheelDebug_flg)  "<VTPM_RRWheelDebug_flg>"
  bus_selector8/44 -> outpmodule/349(VPMM_PwrStaTOSta_enum)  "<VPMM_PwrStaTOSta_enum>"
  bus_selector15/47 -> outpmodule/631(VVMC_ADASForceIdle_flg)  "<VVMC_ADASForceIdle_flg>"
  outpmodule/124(VOUTP_BrkSwVTimeOut_flg) -> bus_creator/124
  outpmodule/493(VOUTP_RFP20_raw8) -> bus_creator/493
  bus_selector8/43 -> outpmodule/348(VPMM_CtrlDrPwrStbA2_flg)  "<VPMM_CtrlDrPwrStbA2_flg>"
  outpmodule/584(VOUTP_ReqV2LIVIPopup_enum) -> bus_creator/584
  bus_selector8/37 -> outpmodule/342(VPMM_LVSilentChrgLv_enum)  "<VPMM_LVSilentChrgLv_enum>"
  bus_selector11/35 -> outpmodule/476(VTPM_RRWheelPSW_raw8)  "<VTPM_RRWheelPSW_raw8>"
  outpmodule/466(VOUTP_LRPressIndi_enum) -> bus_creator/466
  bus_selector9/36 -> outpmodule/389(VSYS_CurrentNmState_enum)  "<VSYS_CurrentNmState_enum>"
  outpmodule/156(VOUTP_DriverSeatBeltCmdTimeOut_flg) -> bus_creator/156
  bus_selector8/35 -> outpmodule/340(VPMM_LVSilentChrgSta_enum)  "<VPMM_LVSilentChrgSta_enum>"
  outpmodule/30(VOUTP_USSStaRML_flg) -> bus_creator/30
  bus_selector3/118 -> outpmodule/283(VBCM_FWasSwSta_enum)  "<VBCM_FWasSwSta_enum>"
  outpmodule/567(VOUTP_RrUdcMin_V) -> bus_creator/567
  bus_selector8/34 -> outpmodule/339(VPMM_PMMAllowECUSleep_flg)  "<VPMM_PMMAllowECUSleep_flg>"
  bus_selector10/17 -> outpmodule/406(VTHC_FDFrRiAPTCHeatPwrCmd_W)  "<VTHC_FDFrRiAPTCHeatPwrCmd_W>"
  outpmodule/582(VOUTP_RrTMTqReq_Nm) -> bus_creator/582
  bus_selector8/31 -> outpmodule/336(VPMM_SilentChkAllowSleep_flg)  "<VPMM_SilentChkAllowSleep_flg>"
  outpmodule/297(VOUTP_CSB_flg) -> bus_creator/297
  bus_selector14/2 -> outpmodule/584(VV2L_ReqV2LIVIPopup_enum)  "<VV2L_ReqV2LIVIPopup_enum>"
  outpmodule/557(VOUTP_RgnAbnorSta_flg) -> bus_creator/557
  outpmodule/220(VOUTP_AmbLightBrightness2_enum) -> bus_creator/220
  bus_selector8/30 -> outpmodule/335(VPMM_LVBattChrgTimeCnt_s)  "<VPMM_LVBattChrgTimeCnt_s>"
  bus_selector8/29 -> outpmodule/334(VPMM_LVChrgHoldTtimer_s)  "<VPMM_LVChrgHoldTtimer_s>"
  outpmodule/457(VOUTP_RRSensorFail_flg) -> bus_creator/457
  outpmodule/65(VOUTP_RFWhlRotDir_enum) -> bus_creator/65
  outpmodule/533(VOUTP_ParkRequest_flg) -> bus_creator/533
  bus_selector9/18 -> outpmodule/371(VSYS_Dash1_cnt)  "<VSYS_Dash1_cnt>"
  bus_selector2/56 -> outpmodule/59(VAPM_LRRawWhlSpeedV_flg)  "<VAPM_LRRawWhlSpeedV_flg>"
  bus_selector8/28 -> outpmodule/333(VPMM_IVIPwrStaONTOPopT_s)  "<VPMM_IVIPwrStaONTOPopT_s>"
  bus_selector11/33 -> outpmodule/474(VTPM_LRWheelPSW_raw8)  "<VTPM_LRWheelPSW_raw8>"
  bus_selector2/78 -> outpmodule/81(VAPM_RFPulseCount_enum)  "<VAPM_RFPulseCount_enum>"
  outpmodule/551(VOUTP_FrEDUSpd_rpm) -> bus_creator/551
  bus_selector8/26 -> outpmodule/331(VPMM_EvccAplusPwrUpReq_flg)  "<VPMM_EvccAplusPwrUpReq_flg>"
  outpmodule/141(VOUTP_AVMParkingmode_enum) -> bus_creator/141
  bus_selector8/25 -> outpmodule/330(VPMM_LVSysErrPwrOutErr_flg)  "<VPMM_LVSysErrPwrOutErr_flg>"
  bus_selector3/58 -> outpmodule/223(VBCM_AmbLightBrightness5_enum)  "<VBCM_AmbLightBrightness5_enum>"
  outpmodule/495(VOUTP_RRP20_raw8) -> bus_creator/495
  outpmodule/285(VOUTP_ActAPSPosn_pct) -> bus_creator/285
  bus_selector9/17 -> outpmodule/370(VSYS_Variation_cnt)  "<VSYS_Variation_cnt>"
  outpmodule/520(VOUTP_WriteChkfinRFID_raw) -> bus_creator/520
  outpmodule/120(VOUTP_MCPressureVTimeOut_flg) -> bus_creator/120
  bus_selector9/16 -> outpmodule/369(VSYS_Country2_cnt)  "<VSYS_Country2_cnt>"
  bus_selector3/93 -> outpmodule/258(VBCM_ATCtrl_enum)  "<VBCM_ATCtrl_enum>"
  bus_selector2/119 -> outpmodule/122(VAPM_BrkSwStaTimeOut_flg)  "<VAPM_BrkSwStaTimeOut_flg>"
  outpmodule/576(VOUTP_SaveRegenMode_enum) -> bus_creator/576
  bus_selector9/15 -> outpmodule/368(VSYS_Country1_cnt)  "<VSYS_Country1_cnt>"
  bus_selector2/79 -> outpmodule/82(VAPM_RFPulseCountTimeOut_flg)  "<VAPM_RFPulseCountTimeOut_flg>"
  outpmodule/464(VOUTP_LFPressIndi_enum) -> bus_creator/464
  bus_selector2/11 -> outpmodule/14(VAPM_PASDFML_cm)  "<VAPM_PASDFML_cm>"
  bus_selector3/104 -> outpmodule/269(VBCM_AmbColorSta3_enum)  "<VBCM_AmbColorSta3_enum>"
  outpmodule/373(VOUTP_Change2_cnt) -> bus_creator/373
  bus_selector2/52 -> outpmodule/55(VAPM_LFRawWhlSpeedV_flg)  "<VAPM_LFRawWhlSpeedV_flg>"
  outpmodule/164(VOUTP_APSRqEPASCtrl_flg) -> bus_creator/164
  bus_selector11/14 -> outpmodule/455(VTPM_RFSensorFail_flg)  "<VTPM_RFSensorFail_flg>"
  bus_selector12/25 -> outpmodule/557(VTQD_RgnAbnorSta_flg)  "<VTQD_RgnAbnorSta_flg>"
  bus_selector7/12 -> outpmodule/305(VNMM_NetworkReq_flg)  "<VNMM_NetworkReq_flg>"
  bus_selector12/24 -> outpmodule/556(VTQD_RrEDUAvailBrkRgnTqV_flg)  "<VTQD_RrEDUAvailBrkRgnTqV_flg>"
  bus_selector12/23 -> outpmodule/555(VTQD_RrEDUSpdValid_flg)  "<VTQD_RrEDUSpdValid_flg>"
  bus_selector8/7 -> outpmodule/312(VPMM_DCDCVoltSetpoint_V)  "<VPMM_DCDCVoltSetpoint_V>"
  outpmodule/15(VOUTP_PASDFCR_cm) -> bus_creator/15
  outpmodule/607(VOUTP_ACCRequiredAccel_mps2) -> bus_creator/607
  bus_selector9/6 -> outpmodule/359(VSYS_CarModel3_cnt)  "<VSYS_CarModel3_cnt>"
  bus_selector9/7 -> outpmodule/360(VSYS_ECU1_cnt)  "<VSYS_ECU1_cnt>"
  bus_selector3/4 -> outpmodule/169(VBCM_AllDoorSW_flg)  "<VBCM_AllDoorSW_flg>"
  bus_selector12/22 -> outpmodule/554(VTQD_FrEDUAvailBrkRgnTqV_flg)  "<VTQD_FrEDUAvailBrkRgnTqV_flg>"
  outpmodule/137(VOUTP_AVMparkingcancel_enum) -> bus_creator/137
  outpmodule/603(VOUTP_AccCalcuPID_mps2) -> bus_creator/603
  outpmodule/295(VOUTP_NMmTxReq_flg) -> bus_creator/295
  bus_selector15/34 -> outpmodule/618(VVMC_ACCVehHoldReq_flg)  "<VVMC_ACCVehHoldReq_flg>"
  bus_selector12/20 -> outpmodule/552(VTQD_RrEDUSpd_rpm)  "<VTQD_RrEDUSpd_rpm>"
  bus_selector12/17 -> outpmodule/549(VTQD_FrEDURolRgnTq_Nm)  "<VTQD_FrEDURolRgnTq_Nm>"
  outpmodule/26(VOUTP_PASAFMR_enum) -> bus_creator/26
  bus_selector12/15 -> outpmodule/547(VTQD_FrEDUActTq_Nm)  "<VTQD_FrEDUActTq_Nm>"
  bus_selector12/38 -> outpmodule/570(VTQD_CreepON_flg)  "<VTQD_CreepON_flg>"
  outpmodule/428(VOUTP_FDRecyAutoCmd_enum) -> bus_creator/428
  bus_selector8/41 -> outpmodule/346(VPMM_CtrlFrEDUINVERTER_flg)  "<VPMM_CtrlFrEDUINVERTER_flg>"
  outpmodule/213(VOUTP_AmbLightBreath1_enum) -> bus_creator/213
  bus_selector12/14 -> outpmodule/546(VTQD_DriverWhlTqDemRr_Nm)  "<VTQD_DriverWhlTqDemRr_Nm>"
  bus_selector12/12 -> outpmodule/544(VTQD_RrRgnDecrSta_flg)  "<VTQD_RrRgnDecrSta_flg>"
  outpmodule/13(VOUTP_PASDFMR_cm) -> bus_creator/13
  bus_selector3/40 -> outpmodule/205(VBCM_RoomLampL_flg)  "<VBCM_RoomLampL_flg>"
  bus_selector12/13 -> outpmodule/545(VTQD_DriverWhlTqDemFr_Nm)  "<VTQD_DriverWhlTqDemFr_Nm>"
  bus_selector12/11 -> outpmodule/543(VTQD_FrRgnDecrSta_flg)  "<VTQD_FrRgnDecrSta_flg>"
  bus_selector12/10 -> outpmodule/542(VTQD_RrActvDmpDisabReq_flg)  "<VTQD_RrActvDmpDisabReq_flg>"
  outpmodule/439(VOUTP_fdefog_flg) -> bus_creator/439
  outpmodule/197(VOUTP_HazardSW_flg) -> bus_creator/197
  bus_selector9/34 -> outpmodule/387(VSYS_WisrBootReason_raw32)  "<VSYS_WisrBootReason_raw32>"
  bus_selector12/9 -> outpmodule/541(VTQD_FrActvDmpDisabReq_flg)  "<VTQD_FrActvDmpDisabReq_flg>"
  outpmodule/119(VOUTP_MCPressureV_bar) -> bus_creator/119
  outpmodule/236(VOUTP_CountAlarm_enum) -> bus_creator/236
  bus_selector12/40 -> outpmodule/572(VTQD_DriveProtEn_flg)  "<VTQD_DriveProtEn_flg>"
  bus_selector3/95 -> outpmodule/260(VBCM_UserNow_enum)  "<VBCM_UserNow_enum>"
  bus_selector12/36 -> outpmodule/568(VTQD_RrUdcMax_V)  "<VTQD_RrUdcMax_V>"
  bus_selector1/3 -> outpmodule/3(VACC_VehHVPwrAvail4THCM_W)  "<VACC_VehHVPwrAvail4THCM_W>"
  bus_selector12/6 -> outpmodule/538(VTQD_EVDriveMode_enum)  "<VTQD_EVDriveMode_enum>"
  bus_selector12/5 -> outpmodule/537(VTQD_RrEDUAvailBrkRgnTq_Nm)  "<VTQD_RrEDUAvailBrkRgnTq_Nm>"
  bus_selector12/4 -> outpmodule/536(VTQD_FrEDUAvailBrkRgnTq_Nm)  "<VTQD_FrEDUAvailBrkRgnTq_Nm>"
  bus_selector12/27 -> outpmodule/559(VTQD_FrRgnPermSta_flg)  "<VTQD_FrRgnPermSta_flg>"
  bus_selector2/31 -> outpmodule/34(VAPM_USSStaRCL_flg)  "<VAPM_USSStaRCL_flg>"
  bus_selector2/96 -> outpmodule/99(VAPM_SASCAL_flg)  "<VAPM_SASCAL_flg>"
  bus_selector12/26 -> outpmodule/558(VTQD_PTCSPermSta_flg)  "<VTQD_PTCSPermSta_flg>"
  outpmodule/540(VOUTP_PButtonSta_enum) -> bus_creator/540
  bus_selector12/1 -> outpmodule/533(VTQD_ParkRequest_flg)  "<VTQD_ParkRequest_flg>"
  bus_selector7/8 -> outpmodule/301(VNMM_RptMsgReq_flg)  "<VNMM_RptMsgReq_flg>"
  outpmodule/57(VOUTP_RFRawWhlSpeedV_flg) -> bus_creator/57
  bus_selector11/91 -> outpmodule/532(VTPM_FlashIDvalid_enum)  "<VTPM_FlashIDvalid_enum>"
  outpmodule/435(VOUTP_CCUSyncSts_flg) -> bus_creator/435
  bus_selector9/11 -> outpmodule/364(VSYS_Minor1_cnt)  "<VSYS_Minor1_cnt>"
  outpmodule/364(VOUTP_Minor1_cnt) -> bus_creator/364
  bus_selector10/18 -> outpmodule/407(VTHC_FDRrAPTCHeatPwrCmd_W)  "<VTHC_FDRrAPTCHeatPwrCmd_W>"
  bus_selector11/90 -> outpmodule/531(VTPM_FlashS4ID_raw)  "<VTPM_FlashS4ID_raw>"
  bus_selector3/56 -> outpmodule/221(VBCM_AmbLightBrightness3_enum)  "<VBCM_AmbLightBrightness3_enum>"
  bus_selector2/97 -> outpmodule/100(VAPM_SASCALTimeOut_flg)  "<VAPM_SASCALTimeOut_flg>"
  bus_selector10/1 -> outpmodule/390(VTHC_FDCompCmd_rpm)  "<VTHC_FDCompCmd_rpm>"
  outpmodule/534(VOUTP_TqSourceFr_enum) -> bus_creator/534
  bus_selector11/89 -> outpmodule/530(VTPM_FlashS3ID_raw)  "<VTPM_FlashS3ID_raw>"
  bus_selector11/88 -> outpmodule/529(VTPM_FlashS2ID_raw)  "<VTPM_FlashS2ID_raw>"
  bus_selector11/84 -> outpmodule/525(VTPM_unlearnSfali_flg)  "<VTPM_unlearnSfali_flg>"
  bus_selector8/19 -> outpmodule/324(VPMM_PwrStaConstraint_enum)  "<VPMM_PwrStaConstraint_enum>"
  BTPM_outputs/1 -> bus_selector11/1
  outpmodule/459(VOUTP_LRWheelDebug_flg) -> bus_creator/459
  bus_selector11/85 -> outpmodule/526(VTPM_unlearnSfailvalid_enum)  "<VTPM_unlearnSfailvalid_enum>"
  bus_selector3/100 -> outpmodule/265(VBCM_AmbPwrWarnENFlash_enum)  "<VBCM_AmbPwrWarnENFlash_enum>"
  bus_selector11/82 -> outpmodule/523(VTPM_Flashchkdatavalid_enum)  "<VTPM_Flashchkdatavalid_enum>"
  outpmodule/118(VOUTP_LongAccelVTimeOut_flg) -> bus_creator/118
  outpmodule/605(VOUTP_ISODecLimit_mps2) -> bus_creator/605
  bus_selector11/81 -> outpmodule/522(VTPM_WriteChkfinRRID_raw)  "<VTPM_WriteChkfinRRID_raw>"
  bus_selector11/80 -> outpmodule/521(VTPM_WriteChkfinLRID_raw)  "<VTPM_WriteChkfinLRID_raw>"
  bus_selector11/78 -> outpmodule/519(VTPM_WriteChkfinLFID_raw)  "<VTPM_WriteChkfinLFID_raw>"
  bus_selector8/32 -> outpmodule/337(VPMM_TimerAllowSleep_flg)  "<VPMM_TimerAllowSleep_flg>"
  bus_selector11/79 -> outpmodule/520(VTPM_WriteChkfinRFID_raw)  "<VTPM_WriteChkfinRFID_raw>"
  bus_selector8/27 -> outpmodule/332(VPMM_PwrStaONTOPopReq_flg)  "<VPMM_PwrStaONTOPopReq_flg>"
  bus_selector2/57 -> outpmodule/60(VAPM_LRRawWhlSpeedVTimeOut_flg)  "<VAPM_LRRawWhlSpeedVTimeOut_flg>"
  bus_selector11/77 -> outpmodule/518(VTPM_WriteChkRRID_raw)  "<VTPM_WriteChkRRID_raw>"
  bus_selector8/36 -> outpmodule/341(VPMM_LVSilentChrgReq_flg)  "<VPMM_LVSilentChrgReq_flg>"
  bus_selector11/76 -> outpmodule/517(VTPM_WriteChkLRID_raw)  "<VTPM_WriteChkLRID_raw>"
  bus_selector11/73 -> outpmodule/514(VTPM_RRPindi_enum)  "<VTPM_RRPindi_enum>"
  bus_selector8/24 -> outpmodule/329(VPMM_ReVehThdChkSta_enum)  "<VPMM_ReVehThdChkSta_enum>"
  outpmodule/536(VOUTP_FrEDUAvailBrkRgnTq_Nm) -> bus_creator/536
  bus_selector11/71 -> outpmodule/512(VTPM_RFPind_enum)  "<VTPM_RFPind_enum>"
  outpmodule/450(VOUTP_LFWheelTemp_C) -> bus_creator/450
  outpmodule/102(VOUTP_SASVTimeOut_flg) -> bus_creator/102
  BTQR_outputs/1 -> bus_selector13/1
  bus_selector11/70 -> outpmodule/511(VTPM_LFPindi_enum)  "<VTPM_LFPindi_enum>"
  bus_selector11/69 -> outpmodule/510(VTPM_TPMSResButt_flg)  "<VTPM_TPMSResButt_flg>"
  bus_selector11/68 -> outpmodule/509(VTPM_ChkStorge_flg)  "<VTPM_ChkStorge_flg>"
  bus_selector8/23 -> outpmodule/328(VPMM_LowSOCWarn_enum)  "<VPMM_LowSOCWarn_enum>"
  bus_selector4/3 -> outpmodule/287(VDHP_EAPS2MIN_pct)  "<VDHP_EAPS2MIN_pct>"
  bus_selector11/67 -> outpmodule/508(VTPM_TPMSStorge_flg)  "<VTPM_TPMSStorge_flg>"
  bus_selector3/11 -> outpmodule/176(VBCM_RLDoorSW_flg)  "<VBCM_RLDoorSW_flg>"
  bus_selector11/66 -> outpmodule/507(VTPM_SetIDLoc_flg)  "<VTPM_SetIDLoc_flg>"
  outpmodule/123(VOUTP_BrkSwV_flg) -> bus_creator/123
  bus_selector15/20 -> outpmodule/604(VVMC_ISOAccLimit_mps2)  "<VVMC_ISOAccLimit_mps2>"
  bus_selector11/62 -> outpmodule/503(VTPM_ID2messageALTU_raw8)  "<VTPM_ID2messageALTU_raw8>"
  bus_selector11/63 -> outpmodule/504(VTPM_ID3messageALTU_raw8)  "<VTPM_ID3messageALTU_raw8>"
  bus_selector2/81 -> outpmodule/84(VAPM_LRPulseCountTimeOut_flg)  "<VAPM_LRPulseCountTimeOut_flg>"
  bus_selector15/25 -> outpmodule/609(VVMC_FeatArbitrFinal_enum)  "<VVMC_FeatArbitrFinal_enum>"
  outpmodule/86(VOUTP_RRPulseCountTimeOut_flg) -> bus_creator/86
  bus_selector11/64 -> outpmodule/505(VTPM_ID4messageALTU_raw8)  "<VTPM_ID4messageALTU_raw8>"
  outpmodule/187(VOUTP_PosLamp_flg) -> bus_creator/187
  outpmodule/446(VOUTP_LFWheelPress_raw8) -> bus_creator/446
  bus_selector1/1 -> outpmodule/1(VACC_HVTHCMSysAvail_enum)  "<VACC_HVTHCMSysAvail_enum>"
  bus_selector11/59 -> outpmodule/500(VTPM_S3WheelDebugALTU_pct)  "<VTPM_S3WheelDebugALTU_pct>"
  outpmodule/177(VOUTP_RRDoorSW_flg) -> bus_creator/177
  outpmodule/178(VOUTP_LockSetting_flg) -> bus_creator/178
  bus_selector11/60 -> outpmodule/501(VTPM_S4WheelDebugALTU_pct)  "<VTPM_S4WheelDebugALTU_pct>"
  outpmodule/202(VOUTP_MirrorDefog_flg) -> bus_creator/202
  bus_selector11/58 -> outpmodule/499(VTPM_S2WheelDebugALTU_pct)  "<VTPM_S2WheelDebugALTU_pct>"
  outpmodule/142(VOUTP_AVMParkingmodeTimeOut_flg) -> bus_creator/142
  bus_selector11/57 -> outpmodule/498(VTPM_S1WheelDebugALTU_pct)  "<VTPM_S1WheelDebugALTU_pct>"
  outpmodule/258(VOUTP_ATCtrl_enum) -> bus_creator/258
  outpmodule/82(VOUTP_RFPulseCountTimeOut_flg) -> bus_creator/82
  bus_selector11/55 -> outpmodule/496(VTPM_FAT_flg)  "<VTPM_FAT_flg>"
  bus_selector11/56 -> outpmodule/497(VTPM_IDin_raw32)  "<VTPM_IDin_raw32>"
  bus_selector8/33 -> outpmodule/338(VPMM_FDADC12VDetAvg_mV)  "<VPMM_FDADC12VDetAvg_mV>"
  outpmodule/83(VOUTP_LRPulseCount_enum) -> bus_creator/83
  bus_selector11/54 -> outpmodule/495(VTPM_RRP20_raw8)  "<VTPM_RRP20_raw8>"
  bus_selector3/63 -> outpmodule/228(VBCM_AmbLightColor4_enum)  "<VBCM_AmbLightColor4_enum>"
  outpmodule/454(VOUTP_LFSensorFail_flg) -> bus_creator/454
  bus_selector11/53 -> outpmodule/494(VTPM_LRP20_raw8)  "<VTPM_LRP20_raw8>"
  bus_selector2/129 -> outpmodule/132(VAPM_EPBExtApplyAvailTimeOut_flg)  "<VAPM_EPBExtApplyAvailTimeOut_flg>"
  bus_selector11/52 -> outpmodule/493(VTPM_RFP20_raw8)  "<VTPM_RFP20_raw8>"
  outpmodule/209(VOUTP_FrWiperH_flg) -> bus_creator/209
  bus_selector8/40 -> outpmodule/345(VPMM_CtrlFrBMSCCUCIR_flg)  "<VPMM_CtrlFrBMSCCUCIR_flg>"
  bus_selector11/51 -> outpmodule/492(VTPM_LFP20_raw8)  "<VTPM_LFP20_raw8>"
  outpmodule/541(VOUTP_FrActvDmpDisabReq_flg) -> bus_creator/541
  outpmodule/204(VOUTP_RoomLampH_flg) -> bus_creator/204
  bus_selector11/50 -> outpmodule/491(VTPM_ALFin_flg)  "<VTPM_ALFin_flg>"
  outpmodule/247(VOUTP_LRRDCtrlCmd_pct) -> bus_creator/247
  outpmodule/589(VOUTP_VMCAEBCtrlAvail_flg) -> bus_creator/589
  bus_selector11/49 -> outpmodule/490(VTPM_S4L_enum)  "<VTPM_S4L_enum>"
  outpmodule/125(VOUTP_ESCStandstill_flg) -> bus_creator/125
  outpmodule/254(VOUTP_AmbODAEN_flg) -> bus_creator/254
  bus_selector11/47 -> outpmodule/488(VTPM_S2L_enum)  "<VTPM_S2L_enum>"
  outpmodule/231(VOUTP_LampPwr_flg) -> bus_creator/231
  outpmodule/572(VOUTP_DriveProtEn_flg) -> bus_creator/572
  bus_selector2/71 -> outpmodule/74(VAPM_RFPulseCountVTimeOut_flg)  "<VAPM_RFPulseCountVTimeOut_flg>"
  outpmodule/116(VOUTP_LatAccelVTimeOut_flg) -> bus_creator/116
  bus_selector2/38 -> outpmodule/41(VAPM_Chime_enum)  "<VAPM_Chime_enum>"
  bus_selector2/40 -> outpmodule/43(VAPM_StaFSya_flg)  "<VAPM_StaFSya_flg>"
  outpmodule/173(VOUTP_TailgateSW_flg) -> bus_creator/173
  bus_selector15/56 -> outpmodule/640(VVMC_ACCTakeoverReq_flg)  "<VVMC_ACCTakeoverReq_flg>"
  outpmodule/472(VOUTP_RRWheelTmpIndi_flg) -> bus_creator/472
  bus_selector3/30 -> outpmodule/195(VBCM_LBSD_flg)  "<VBCM_LBSD_flg>"
  outpmodule/685(VOUTP_VMCRWSPositionReq_mm) -> bus_creator/685
  outpmodule/686(VOUTP_VMCSteerFaultRequest_enum) -> bus_creator/686
  outpmodule/683(VOUTP_VMCRWSActvSta_enum) -> bus_creator/683
  bus_selector8/38 -> outpmodule/343(VPMM_CtrlFrPwrStbA1P_flg)  "<VPMM_CtrlFrPwrStbA1P_flg>"
  outpmodule/684(VOUTP_VMCRWSDfctvSta_enum) -> bus_creator/684
  bus_selector2/126 -> outpmodule/129(VAPM_EPBExtReleaseAvail_flg)  "<VAPM_EPBExtReleaseAvail_flg>"
  outpmodule/680(VOUTP_IMUEnaCmd_flg) -> bus_creator/680
  bus_selector12/3 -> outpmodule/535(VTQD_TqSourceRr_enum)  "<VTQD_TqSourceRr_enum>"
  outpmodule/682(VOUTP_CAASActive_flg) -> bus_creator/682
  bus_selector11/48 -> outpmodule/489(VTPM_S3L_enum)  "<VTPM_S3L_enum>"
  outpmodule/681(VOUTP_CAASCtrlAvail_flg) -> bus_creator/681
  outpmodule/233(VOUTP_APSOpenPTG_flg) -> bus_creator/233
  outpmodule/678(VOUTP_APSReq_enum) -> bus_creator/678
  bus_selector3/74 -> outpmodule/239(VBCM_FuelDoorPos_flg)  "<VBCM_FuelDoorPos_flg>"
  outpmodule/101(VOUTP_SASV_flg) -> bus_creator/101
  outpmodule/679(VOUTP_CCMSASpdWar_flg) -> bus_creator/679
  bus_selector12/7 -> outpmodule/539(VTQD_ShiftGearPosn_enum)  "<VTQD_ShiftGearPosn_enum>"
  bus_selector3/17 -> outpmodule/182(VBCM_CTDCtrl_enum)  "<VBCM_CTDCtrl_enum>"
  outpmodule/675(VOUTP_APSStaSys_enum) -> bus_creator/675
  bus_selector10/5 -> outpmodule/394(VTHC_FDEXV1Cmd_step)  "<VTHC_FDEXV1Cmd_step>"
  bus_selector12/16 -> outpmodule/548(VTQD_RrEDUActTq_Nm)  "<VTQD_RrEDUActTq_Nm>"
  outpmodule/676(VOUTP_APSDecReqA_flg) -> bus_creator/676
  outpmodule/677(VOUTP_APSDecReq_mps2) -> bus_creator/677
  outpmodule/674(VOUTP_APSCtrlAvail_flg) -> bus_creator/674
  bus_selector12/8 -> outpmodule/540(VTQD_PButtonSta_enum)  "<VTQD_PButtonSta_enum>"
  outpmodule/64(VOUTP_LFWhlRotDirTimeOut_flg) -> bus_creator/64
  outpmodule/378(VOUTP_SHA4_cnt) -> bus_creator/378
  outpmodule/673(VOUTP_MSACtrlSta_enum) -> bus_creator/673
  outpmodule/672(VOUTP_CCCtrlSta_enum) -> bus_creator/672
  bus_selector2/67 -> outpmodule/70(VAPM_RRWhlRotDirTimeOut_flg)  "<VAPM_RRWhlRotDirTimeOut_flg>"
  outpmodule/28(VOUTP_PASAFCR_enum) -> bus_creator/28
  outpmodule/670(VOUTP_ACCPedalOvrd_flg) -> bus_creator/670
  outpmodule/669(VOUTP_ACCCtrlAvail_flg) -> bus_creator/669
  bus_selector3/67 -> outpmodule/232(VBCM_SPTGDet_flg)  "<VBCM_SPTGDet_flg>"
  bus_selector2/60 -> outpmodule/63(VAPM_LFWhlRotDir_enum)  "<VAPM_LFWhlRotDir_enum>"
  outpmodule/367(VOUTP_Patch2_cnt) -> bus_creator/367
  outpmodule/668(VOUTP_FCMLDWFault_flg) -> bus_creator/668
  outpmodule/666(VOUTP_ADASAEBSta_enum) -> bus_creator/666
  bus_selector12/44 -> outpmodule/576(VTQD_SaveRegenMode_enum)  "<VTQD_SaveRegenMode_enum>"
  outpmodule/31(VOUTP_USSStaRLR_flg) -> bus_creator/31
  bus_selector9/1 -> outpmodule/354(VSYS_HWVer1_cnt)  "<VSYS_HWVer1_cnt>"
  outpmodule/537(VOUTP_RrEDUAvailBrkRgnTq_Nm) -> bus_creator/537
  bus_selector12/39 -> outpmodule/571(VTQD_EquivAccPedalSWSta_flg)  "<VTQD_EquivAccPedalSWSta_flg>"
  outpmodule/667(VOUTP_FCMLDWRequest_enum) -> bus_creator/667
  bus_selector2/95 -> outpmodule/98(VAPM_SASSpeedValidTimeOut_flg)  "<VAPM_SASSpeedValidTimeOut_flg>"
  outpmodule/663(VOUTP_ADASLanetypeL_enum) -> bus_creator/663
  outpmodule/22(VOUTP_PASARMR_enum) -> bus_creator/22
  outpmodule/665(VOUTP_ADASLanecurveR_raw32) -> bus_creator/665
  outpmodule/356(VOUTP_HWVer3_cnt) -> bus_creator/356
  bus_selector10/39 -> outpmodule/428(VTHC_FDRecyAutoCmd_enum)  "<VTHC_FDRecyAutoCmd_enum>"
  outpmodule/507(VOUTP_SetIDLoc_flg) -> bus_creator/507
  bus_selector2/34 -> outpmodule/37(VAPM_USSStaFLR_flg)  "<VAPM_USSStaFLR_flg>"
  outpmodule/62(VOUTP_RRRawWhlSpeedVTimeOut_flg) -> bus_creator/62
  bus_selector6/3 -> outpmodule/292(VDSC_DISCSta_enum)  "<VDSC_DISCSta_enum>"
  bus_selector15/98 -> outpmodule/682(VVMC_CAASActive_flg)  "<VVMC_CAASActive_flg>"
  outpmodule/664(VOUTP_ADASLanecurveL_raw32) -> bus_creator/664
  outpmodule/207(VOUTP_TailgateHDSW_flg) -> bus_creator/207
  outpmodule/662(VOUTP_ADASLanetypeR_enum) -> bus_creator/662
  bus_selector2/90 -> outpmodule/93(VAPM_SASAngle_Deg)  "<VAPM_SASAngle_Deg>"
  bus_selector3/114 -> outpmodule/279(VBCM_HazardIND_flg)  "<VBCM_HazardIND_flg>"
  outpmodule/661(VOUTP_FCMACCmode_enum) -> bus_creator/661
  outpmodule/372(VOUTP_Change1_cnt) -> bus_creator/372
  outpmodule/658(VOUTP_LVDAWarning_flg) -> bus_creator/658
  bus_selector8/21 -> outpmodule/326(VPMM_PwrUpReq_enum)  "<VPMM_PwrUpReq_enum>"
  outpmodule/660(VOUTP_ADASLFCWarnSound_enum) -> bus_creator/660
  bus_selector15/96 -> outpmodule/680(VVMC_IMUEnaCmd_flg)  "<VVMC_IMUEnaCmd_flg>"
  bus_selector11/61 -> outpmodule/502(VTPM_ID1messageALTU_raw8)  "<VTPM_ID1messageALTU_raw8>"
  bus_selector3/41 -> outpmodule/206(VBCM_TrunkRel_flg)  "<VBCM_TrunkRel_flg>"
  bus_selector3/103 -> outpmodule/268(VBCM_AmbColorSta2_enum)  "<VBCM_AmbColorSta2_enum>"
  outpmodule/8(VOUTP_ChrgPlugSta_enum) -> bus_creator/8
  outpmodule/659(VOUTP_LVDAACCStatusInformation_flg) -> bus_creator/659
  outpmodule/657(VOUTP_LVDAFailinfo_flg) -> bus_creator/657
  bus_selector2/123 -> outpmodule/126(VAPM_ESCStandstillTimeOut_flg)  "<VAPM_ESCStandstillTimeOut_flg>"
  outpmodule/656(VOUTP_LVDAMuteSta_enum) -> bus_creator/656
  bus_selector10/48 -> outpmodule/437(VTHC_RecAutoFlg_flg)  "<VTHC_RecAutoFlg_flg>"
  bus_selector2/148 -> outpmodule/151(VAPM_ABSActive_flg)  "<VAPM_ABSActive_flg>"
  outpmodule/654(VOUTP_ADASLFCHandsOffWarning_enum) -> bus_creator/654
  outpmodule/655(VOUTP_LVDADisabled_flg) -> bus_creator/655
  outpmodule/653(VOUTP_ADASFCWMute_flg) -> bus_creator/653
  bus_selector15/90 -> outpmodule/674(VVMC_APSCtrlAvail_flg)  "<VVMC_APSCtrlAvail_flg>"
  BACC_outputs/1 -> bus_selector1/1
  outpmodule/650(VOUTP_ADASSLIFSta_enum) -> bus_creator/650
  outpmodule/651(VOUTP_ADASISASta_enum) -> bus_creator/651
  bus_selector2/15 -> outpmodule/18(VAPM_APSDRLL_cm)  "<VAPM_APSDRLL_cm>"
  outpmodule/649(VOUTP_ADASLaneModeR_enum) -> bus_creator/649
  bus_selector3/91 -> outpmodule/256(VBCM_AmbBrightSta_enum)  "<VBCM_AmbBrightSta_enum>"
  outpmodule/647(VOUTP_ADASLFCSta_enum) -> bus_creator/647
  outpmodule/153(VOUTP_TCSActive_flg) -> bus_creator/153
  outpmodule/644(VOUTP_ADASSLIFSpdLim_enum) -> bus_creator/644
  outpmodule/492(VOUTP_LFP20_raw8) -> bus_creator/492
  bus_selector11/87 -> outpmodule/528(VTPM_FlashS1ID_raw)  "<VTPM_FlashS1ID_raw>"
  outpmodule/642(VOUTP_ADASCAMSpdLim_enum) -> bus_creator/642
  outpmodule/362(VOUTP_Major1_cnt) -> bus_creator/362
  outpmodule/485(VOUTP_S3ID_raw32) -> bus_creator/485
  outpmodule/2(VOUTP_LVBattVoltSta_enum) -> bus_creator/2
  outpmodule/640(VOUTP_ACCTakeoverReq_flg) -> bus_creator/640
  bus_selector11/2 -> outpmodule/443(VTPM_RFBatWarn_flg)  "<VTPM_RFBatWarn_flg>"
  bus_selector12/21 -> outpmodule/553(VTQD_FrEDUSpdValid_flg)  "<VTQD_FrEDUSpdValid_flg>"
  outpmodule/79(VOUTP_LFPulseCount_enum) -> bus_creator/79
  outpmodule/641(VOUTP_ADASWarningMsg_enum) -> bus_creator/641
  outpmodule/253(VOUTP_AmbPwrWarnEN_flg) -> bus_creator/253
  outpmodule/637(VOUTP_ADASFltWrnReq_flg) -> bus_creator/637
  bus_selector2/63 -> outpmodule/66(VAPM_RFWhlRotDirTimeOut_flg)  "<VAPM_RFWhlRotDirTimeOut_flg>"
  outpmodule/468(VOUTP_TPMSWarnIndi_enum) -> bus_creator/468
  outpmodule/51(VOUTP_LRRawWhlSpeed_kph) -> bus_creator/51
  outpmodule/633(VOUTP_RightTurnLightReq_flg) -> bus_creator/633
  outpmodule/646(VOUTP_LKAHODSoundWarning_flg) -> bus_creator/646
  outpmodule/632(VOUTP_HazardWarningReq_flg) -> bus_creator/632
  bus_selector15/2 -> outpmodule/586(VVMC_VehicleSpeed_mph)  "<VVMC_VehicleSpeed_mph>"
  bus_selector8/39 -> outpmodule/344(VPMM_CtrlFrRC1_flg)  "<VPMM_CtrlFrRC1_flg>"
  bus_selector11/40 -> outpmodule/481(VTPM_LRSensorMode_flg)  "<VTPM_LRSensorMode_flg>"
  outpmodule/630(VOUTP_ADASShftPosnReq_enum) -> bus_creator/630
  outpmodule/474(VOUTP_LRWheelPSW_raw8) -> bus_creator/474
  outpmodule/349(VOUTP_PwrStaTOSta_enum) -> bus_creator/349
  bus_selector2/111 -> outpmodule/114(VAPM_YawRateVTimeOut_flg)  "<VAPM_YawRateVTimeOut_flg>"
  bus_selector2/48 -> outpmodule/51(VAPM_LRRawWhlSpeed_kph)  "<VAPM_LRRawWhlSpeed_kph>"
  outpmodule/639(VOUTP_ForceLowBeam_enum) -> bus_creator/639
  outpmodule/629(VOUTP_ADASShftPosnReqA_flg) -> bus_creator/629
  bus_selector11/83 -> outpmodule/524(VTPM_Flashdatavalid_enum)  "<VTPM_Flashdatavalid_enum>"
  outpmodule/626(VOUTP_ACCJerkLowerLimit_mps3) -> bus_creator/626
  outpmodule/628(VOUTP_ADASVehSpdLim_raw32) -> bus_creator/628
  outpmodule/638(VOUTP_ACCObjDstLvl_enum) -> bus_creator/638
  outpmodule/625(VOUTP_ACCComfortBandUpper_mps2) -> bus_creator/625
  bus_selector3/75 -> outpmodule/240(VBCM_MFRDNBrightReq_pct)  "<VBCM_MFRDNBrightReq_pct>"
  outpmodule/516(VOUTP_WriteChkRFID_raw) -> bus_creator/516
  outpmodule/315(VOUTP_PowerSta_enum) -> bus_creator/315
  bus_selector2/110 -> outpmodule/113(VAPM_YawRateV_flg)  "<VAPM_YawRateV_flg>"
  outpmodule/623(VOUTP_TimeGapLevel_enum) -> bus_creator/623
  outpmodule/163(VOUTP_APSVRqEPASCtrl_flg) -> bus_creator/163
  outpmodule/627(VOUTP_ACCComfortBandLower_mps2) -> bus_creator/627
  bus_selector2/132 -> outpmodule/135(VAPM_EPBSta_enum)  "<VAPM_EPBSta_enum>"
  outpmodule/167(VOUTP_TailgateRemote_enum) -> bus_creator/167
  bus_selector11/75 -> outpmodule/516(VTPM_WriteChkRFID_raw)  "<VTPM_WriteChkRFID_raw>"
  bus_selector11/41 -> outpmodule/482(VTPM_RRSensorMode_flg)  "<VTPM_RRSensorMode_flg>"
  outpmodule/622(VOUTP_ACCObjRelSpd_mps) -> bus_creator/622
  outpmodule/74(VOUTP_RFPulseCountVTimeOut_flg) -> bus_creator/74
  outpmodule/344(VOUTP_CtrlFrRC1_flg) -> bus_creator/344
  bus_selector2/145 -> outpmodule/148(VAPM_CAASSwTimeOut_flg)  "<VAPM_CAASSwTimeOut_flg>"
  bus_selector12/34 -> outpmodule/566(VTQD_RrIdcMax_A)  "<VTQD_RrIdcMax_A>"
  outpmodule/45(VOUTP_BrkPedalPos_pct) -> bus_creator/45
  outpmodule/469(VOUTP_LFWheelTmpIndi_flg) -> bus_creator/469
  bus_selector12/32 -> outpmodule/564(VTQD_FrUdcMax_V)  "<VTQD_FrUdcMax_V>"
  outpmodule/671(VOUTP_TimeGapCalcu_s) -> bus_creator/671
  bus_selector12/29 -> outpmodule/561(VTQD_FrIdcMin_A)  "<VTQD_FrIdcMin_A>"
  outpmodule/405(VOUTP_FDFrLeAPTCHeatPwrCmd_W) -> bus_creator/405
  bus_selector11/72 -> outpmodule/513(VTPM_LRPindi_enum)  "<VTPM_LRPindi_enum>"
  bus_selector2/104 -> outpmodule/107(VAPM_LatAccel_Gps)  "<VAPM_LatAccel_Gps>"
  bus_selector12/28 -> outpmodule/560(VTQD_RrRgnPermSta_flg)  "<VTQD_RrRgnPermSta_flg>"
  outpmodule/503(VOUTP_ID2messageALTU_raw8) -> bus_creator/503
  outpmodule/221(VOUTP_AmbLightBrightness3_enum) -> bus_creator/221
  bus_selector12/30 -> outpmodule/562(VTQD_FrIdcMax_A)  "<VTQD_FrIdcMax_A>"
  outpmodule/631(VOUTP_ADASForceIdle_flg) -> bus_creator/631
  outpmodule/337(VOUTP_TimerAllowSleep_flg) -> bus_creator/337
  bus_selector11/13 -> outpmodule/454(VTPM_LFSensorFail_flg)  "<VTPM_LFSensorFail_flg>"
  outpmodule/306(VOUTP_PowerUpState_enum) -> bus_creator/306
  outpmodule/336(VOUTP_SilentChkAllowSleep_flg) -> bus_creator/336
  outpmodule/335(VOUTP_LVBattChrgTimeCnt_s) -> bus_creator/335
  outpmodule/96(VOUTP_SASSpeedTimeOut_flg) -> bus_creator/96
  outpmodule/339(VOUTP_PMMAllowECUSleep_flg) -> bus_creator/339
  outpmodule/206(VOUTP_TrunkRel_flg) -> bus_creator/206
  outpmodule/599(VOUTP_SingleWhlSlipRatioCtrl_flg) -> bus_creator/599
  bus_selector11/36 -> outpmodule/477(VTPM_CWheelTips_enum)  "<VTPM_CWheelTips_enum>"
  bus_selector2/86 -> outpmodule/89(VAPM_DriIntend_enum)  "<VAPM_DriIntend_enum>"
  outpmodule/376(VOUTP_SHA2_cnt) -> bus_creator/376
  bus_selector9/19 -> outpmodule/372(VSYS_Change1_cnt)  "<VSYS_Change1_cnt>"
  outpmodule/162(VOUTP_APSAngleTarget_Deg) -> bus_creator/162
  bus_selector9/28 -> outpmodule/381(VSYS_SHA7_cnt)  "<VSYS_SHA7_cnt>"
  bus_selector2/47 -> outpmodule/50(VAPM_RFRawWhlSpeedTimeOut_flg)  "<VAPM_RFRawWhlSpeedTimeOut_flg>"
  outpmodule/135(VOUTP_EPBSta_enum) -> bus_creator/135
  outpmodule/391(VOUTP_FDSOV1Cmd_flg) -> bus_creator/391
  outpmodule/140(VOUTP_AVMparkingexcuteTimeOut_flg) -> bus_creator/140
  bus_selector12/31 -> outpmodule/563(VTQD_FrUdcMin_V)  "<VTQD_FrUdcMin_V>"
  outpmodule/410(VOUTP_EDriveMode_enum) -> bus_creator/410
  bus_selector11/74 -> outpmodule/515(VTPM_WriteChkLFID_raw)  "<VTPM_WriteChkLFID_raw>"
  outpmodule/635(VOUTP_ADASFCWSta_enum) -> bus_creator/635
  outpmodule/553(VOUTP_FrEDUSpdValid_flg) -> bus_creator/553
  bus_selector9/27 -> outpmodule/380(VSYS_SHA6_cnt)  "<VSYS_SHA6_cnt>"
  bus_selector9/26 -> outpmodule/379(VSYS_SHA5_cnt)  "<VSYS_SHA5_cnt>"
  bus_selector12/2 -> outpmodule/534(VTQD_TqSourceFr_enum)  "<VTQD_TqSourceFr_enum>"
  bus_selector9/25 -> outpmodule/378(VSYS_SHA4_cnt)  "<VSYS_SHA4_cnt>"
  bus_selector2/65 -> outpmodule/68(VAPM_LRWhlRotDirTimeOut_flg)  "<VAPM_LRWhlRotDirTimeOut_flg>"
  outpmodule/46(VOUTP_BrkPedalPosTimeOut_flg) -> bus_creator/46
  bus_selector12/33 -> outpmodule/565(VTQD_RrIdcMin_A)  "<VTQD_RrIdcMin_A>"
  bus_selector3/102 -> outpmodule/267(VBCM_AmbColorSta1_enum)  "<VBCM_AmbColorSta1_enum>"
  bus_selector11/65 -> outpmodule/506(VTPM_Chkfin_flg)  "<VTPM_Chkfin_flg>"
  outpmodule/648(VOUTP_ADASLaneModeL_enum) -> bus_creator/648
  bus_selector9/5 -> outpmodule/358(VSYS_CarModel2_cnt)  "<VSYS_CarModel2_cnt>"
  bus_selector9/23 -> outpmodule/376(VSYS_SHA2_cnt)  "<VSYS_SHA2_cnt>"
  bus_selector12/19 -> outpmodule/551(VTQD_FrEDUSpd_rpm)  "<VTQD_FrEDUSpd_rpm>"
  outpmodule/132(VOUTP_EPBExtApplyAvailTimeOut_flg) -> bus_creator/132
  outpmodule/408(VOUTP_FDBlowerCmd_pct) -> bus_creator/408
  outpmodule/338(VOUTP_FDADC12VDetAvg_mV) -> bus_creator/338
  outpmodule/360(VOUTP_ECU1_cnt) -> bus_creator/360
  bus_selector2/114 -> outpmodule/117(VAPM_LongAccelV_flg)  "<VAPM_LongAccelV_flg>"
  outpmodule/278(VOUTP_AmbBrightnessSta7_enum) -> bus_creator/278
  outpmodule/643(VOUTP_TargetType_enum) -> bus_creator/643
  bus_selector2/155 -> outpmodule/158(VAPM_APSRQDisplay_enum)  "<VAPM_APSRQDisplay_enum>"
  bus_selector12/35 -> outpmodule/567(VTQD_RrUdcMin_V)  "<VTQD_RrUdcMin_V>"
  bus_selector2/89 -> outpmodule/92(VAPM_EPSAOIControlTimeOut_flg)  "<VAPM_EPSAOIControlTimeOut_flg>"
  outpmodule/624(VOUTP_ACCJerkUpperLimit_mps3) -> bus_creator/624
  outpmodule/81(VOUTP_RFPulseCount_enum) -> bus_creator/81
  outpmodule/634(VOUTP_LeftTurnLightReq_flg) -> bus_creator/634
  outpmodule/496(VOUTP_FAT_flg) -> bus_creator/496
  outpmodule/268(VOUTP_AmbColorSta2_enum) -> bus_creator/268
  bus_selector9/24 -> outpmodule/377(VSYS_SHA3_cnt)  "<VSYS_SHA3_cnt>"
  outpmodule/84(VOUTP_LRPulseCountTimeOut_flg) -> bus_creator/84
  outpmodule/462(VOUTP_TPMSResButtAllow_flg) -> bus_creator/462
  bus_selector9/22 -> outpmodule/375(VSYS_SHA1_cnt)  "<VSYS_SHA1_cnt>"
  bus_selector15/35 -> outpmodule/619(VVMC_ADASDBSReq_enum)  "<VVMC_ADASDBSReq_enum>"
  outpmodule/147(VOUTP_CAASSw_enum) -> bus_creator/147
  outpmodule/368(VOUTP_Country1_cnt) -> bus_creator/368
  outpmodule/109(VOUTP_LongAccel_Gps) -> bus_creator/109
  bus_selector2/39 -> outpmodule/42(VAPM_SNSRLayout_enum)  "<VAPM_SNSRLayout_enum>"
  outpmodule/645(VOUTP_LKAHODDisplayWarning_flg) -> bus_creator/645
  outpmodule/497(VOUTP_IDin_raw32) -> bus_creator/497
  outpmodule/397(VOUTP_FDFWVCmd_flg) -> bus_creator/397
  bus_selector2/26 -> outpmodule/29(VAPM_USSStaRMR_flg)  "<VAPM_USSStaRMR_flg>"
  bus_selector2/146 -> outpmodule/149(VAPM_IVIScreen_enum)  "<VAPM_IVIScreen_enum>"
  bus_selector2/27 -> outpmodule/30(VAPM_USSStaRML_flg)  "<VAPM_USSStaRML_flg>"
  bus_selector2/24 -> outpmodule/27(VAPM_PASAFML_enum)  "<VAPM_PASAFML_enum>"
  outpmodule/437(VOUTP_RecAutoFlg_flg) -> bus_creator/437
  outpmodule/148(VOUTP_CAASSwTimeOut_flg) -> bus_creator/148
  bus_selector15/6 -> outpmodule/590(VVMC_VMCACCCtrlAvail_flg)  "<VVMC_VMCACCCtrlAvail_flg>"
  bus_selector12/18 -> outpmodule/550(VTQD_RrEDURolRgnTq_Nm)  "<VTQD_RrEDURolRgnTq_Nm>"
  outpmodule/34(VOUTP_USSStaRCL_flg) -> bus_creator/34
  bus_selector9/20 -> outpmodule/373(VSYS_Change2_cnt)  "<VSYS_Change2_cnt>"
  outpmodule/652(VOUTP_ADASLDWMute_flg) -> bus_creator/652
  bus_selector2/25 -> outpmodule/28(VAPM_PASAFCR_enum)  "<VAPM_PASAFCR_enum>"
  bus_selector3/98 -> outpmodule/263(VBCM_AmbDimENFlash_enum)  "<VBCM_AmbDimENFlash_enum>"
  bus_selector2/35 -> outpmodule/38(VAPM_USSStaFLL_flg)  "<VAPM_USSStaFLL_flg>"
  outpmodule/58(VOUTP_RFRawWhlSpeedVTimeOut_flg) -> bus_creator/58
  outpmodule/329(VOUTP_ReVehThdChkSta_enum) -> bus_creator/329
  outpmodule/636(VOUTP_ADASLDWSta_enum) -> bus_creator/636
  bus_selector2/30 -> outpmodule/33(VAPM_USSStaRCR_flg)  "<VAPM_USSStaRCR_flg>"
  bus_selector11/86 -> outpmodule/527(VTPM_Prepresstempvalid_enum)  "<VTPM_Prepresstempvalid_enum>"
  outpmodule/39(VOUTP_USSStaFCR_flg) -> bus_creator/39
  bus_selector2/29 -> outpmodule/32(VAPM_USSStaRLL_flg)  "<VAPM_USSStaRLL_flg>"
  bus_selector12/37 -> outpmodule/569(VTQD_ReBrakeLPReq_flg)  "<VTQD_ReBrakeLPReq_flg>"
  bus_selector2/154 -> outpmodule/157(VAPM_APSProgressPCT_pct)  "<VAPM_APSProgressPCT_pct>"
  outpmodule/583(VOUTP_ReqOBCV2LEna_enum) -> bus_creator/583
  bus_selector9/21 -> outpmodule/374(VSYS_Dash2_cnt)  "<VSYS_Dash2_cnt>"
  bus_selector9/33 -> outpmodule/386(VSYS_PmicBootReason_enum)  "<VSYS_PmicBootReason_enum>"
